simulink model "manul_model_stage15_complete_pre_engineering_20260816"  (R2025a)
settings: Solver=ode3  StartTime=0.0  StopTime=0.3  FixedStep=Ts_power  RelTol=1e-3
InitFcn:
  | run('D:/PV_MPPT/PV_ESS_MPC_Manul_Reproduction/experiments/stage15_bus_stability_20260814/pvess_stage15_busfix_init.m')
values from neighbouring files (symbols this model uses):
  Ad_mpvc = expm(A_mpvc*Ts_mpc)    [pvess_beginner_init_baseline.m]    (also in pvess_stage15_busfix_init.m; pvess_stage15_busfix_init_pre_cpl_20260817.m; pvess_stage15_busfix_init_pre_engineering_20260816.m; pvess_stage15_busfix_init_pre_gridpi_tuning_20260817.m)
  Bd_mpvc = A_mpvc\((Ad_mpvc-eye(2))*B_mpvc)    [pvess_beginner_init_baseline.m]    (also in pvess_stage15_busfix_init.m; pvess_stage15_busfix_init_pre_cpl_20260817.m; pvess_stage15_busfix_init_pre_engineering_20260816.m; pvess_stage15_busfix_init_pre_gridpi_tuning_20260817.m)
  Cdc = 18e-3    (= 0.018)    [pvess_beginner_init_baseline.m]    (also in pvess_stage15_busfix_init.m; pvess_stage15_busfix_init_pre_cpl_20260817.m; pvess_stage15_busfix_init_pre_engineering_20260816.m; pvess_stage15_busfix_init_pre_gridpi_tuning_20260817.m)
  Cpv = 10e-3    (= 0.01)    [pvess_beginner_init_baseline.m]    (also in pvess_stage15_busfix_init.m; pvess_stage15_busfix_init_pre_cpl_20260817.m; pvess_stage15_busfix_init_pre_engineering_20260816.m; pvess_stage15_busfix_init_pre_gridpi_tuning_20260817.m)
  Db0 = 1 - V_bat_nom/Vdc_ref    (= 0.75)    [pvess_beginner_init_baseline.m]    (also in pvess_stage15_busfix_init.m; pvess_stage15_busfix_init_pre_cpl_20260817.m; pvess_stage15_busfix_init_pre_engineering_20260816.m; pvess_stage15_busfix_init_pre_gridpi_tuning_20260817.m)
  Db_max = 0.95    [pvess_beginner_init_baseline.m]    (also in pvess_stage15_busfix_init.m; pvess_stage15_busfix_init_pre_cpl_20260817.m; pvess_stage15_busfix_init_pre_engineering_20260816.m; pvess_stage15_busfix_init_pre_gridpi_tuning_20260817.m)
  Db_min = 0.05    [pvess_beginner_init_baseline.m]    (also in pvess_stage15_busfix_init.m; pvess_stage15_busfix_init_pre_cpl_20260817.m; pvess_stage15_busfix_init_pre_engineering_20260816.m; pvess_stage15_busfix_init_pre_gridpi_tuning_20260817.m)
  Dpv0 = 1 - 547/Vdc_ref    (= 0.544166666667)    [pvess_beginner_init_baseline.m]    (also in pvess_stage15_busfix_init.m; pvess_stage15_busfix_init_pre_cpl_20260817.m; pvess_stage15_busfix_init_pre_engineering_20260816.m; pvess_stage15_busfix_init_pre_gridpi_tuning_20260817.m)
  Dpv_curtail_bias = 0.506    [pvess_stage15_busfix_init.m]    (also in pvess_stage15_busfix_init_pre_cpl_20260817.m; pvess_stage15_busfix_init_pre_engineering_20260816.m; pvess_stage15_busfix_init_pre_gridpi_tuning_20260817.m)
  Dpv_max = 0.75    [pvess_beginner_init_baseline.m]    (also in pvess_stage15_busfix_init.m; pvess_stage15_busfix_init_pre_cpl_20260817.m; pvess_stage15_busfix_init_pre_engineering_20260816.m; pvess_stage15_busfix_init_pre_gridpi_tuning_20260817.m)
  Dpv_min = 0.35    [pvess_beginner_init_baseline.m]    (also in pvess_stage15_busfix_init.m; pvess_stage15_busfix_init_pre_cpl_20260817.m; pvess_stage15_busfix_init_pre_engineering_20260816.m; pvess_stage15_busfix_init_pre_gridpi_tuning_20260817.m)
  Dpv_slew_down = -5.0    (= -5)    [pvess_stage15_busfix_init.m]    (also in pvess_stage15_busfix_init_pre_cpl_20260817.m; pvess_stage15_busfix_init_pre_engineering_20260816.m; pvess_stage15_busfix_init_pre_gridpi_tuning_20260817.m)
  Dpv_slew_up = 1.0    (= 1)    [pvess_stage15_busfix_init.m]    (also in pvess_stage15_busfix_init_pre_cpl_20260817.m; pvess_stage15_busfix_init_pre_engineering_20260816.m; pvess_stage15_busfix_init_pre_gridpi_tuning_20260817.m)
  Dpv_step = 2e-4    (= 0.0002)    [pvess_beginner_init_baseline.m]    (also in pvess_stage15_busfix_init.m; pvess_stage15_busfix_init_pre_cpl_20260817.m; pvess_stage15_busfix_init_pre_engineering_20260816.m; pvess_stage15_busfix_init_pre_gridpi_tuning_20260817.m)
  eps_dI = 1e-3    (= 0.001)    [pvess_beginner_init_baseline.m]    (also in pvess_stage15_busfix_init.m; pvess_stage15_busfix_init_pre_cpl_20260817.m; pvess_stage15_busfix_init_pre_engineering_20260816.m; pvess_stage15_busfix_init_pre_gridpi_tuning_20260817.m)
  eps_dV = 1e-3    (= 0.001)    [pvess_beginner_init_baseline.m]    (also in pvess_stage15_busfix_init.m; pvess_stage15_busfix_init_pre_cpl_20260817.m; pvess_stage15_busfix_init_pre_engineering_20260816.m; pvess_stage15_busfix_init_pre_gridpi_tuning_20260817.m)
  eps_inc = 1e-4    (= 0.0001)    [pvess_beginner_init_baseline.m]    (also in pvess_stage15_busfix_init.m; pvess_stage15_busfix_init_pre_cpl_20260817.m; pvess_stage15_busfix_init_pre_engineering_20260816.m; pvess_stage15_busfix_init_pre_gridpi_tuning_20260817.m)
  f_grid = 50    [pvess_beginner_init_baseline.m]    (also in pvess_stage15_busfix_init.m; pvess_stage15_busfix_init_pre_cpl_20260817.m; pvess_stage15_busfix_init_pre_engineering_20260816.m; pvess_stage15_busfix_init_pre_gridpi_tuning_20260817.m)
  freq_threshold = 0.15    [pvess_beginner_init_baseline.m]    (also in pvess_stage15_busfix_init.m; pvess_stage15_busfix_init_pre_cpl_20260817.m; pvess_stage15_busfix_init_pre_engineering_20260816.m; pvess_stage15_busfix_init_pre_gridpi_tuning_20260817.m)
  Ibat_curtail_release = -0.8*Ibat_max    (= -1333.33333333)    [pvess_stage15_busfix_init.m]    (also in pvess_stage15_busfix_init_pre_cpl_20260817.m; pvess_stage15_busfix_init_pre_engineering_20260816.m; pvess_stage15_busfix_init_pre_gridpi_tuning_20260817.m)
  Ibat_max = P_bat_rated/V_bat_nom    (= 1666.66666667)    [pvess_beginner_init_baseline.m]    (also in pvess_stage15_busfix_init.m; pvess_stage15_busfix_init_pre_cpl_20260817.m; pvess_stage15_busfix_init_pre_engineering_20260816.m; pvess_stage15_busfix_init_pre_gridpi_tuning_20260817.m)
  K_bat_sign = 1    [pvess_beginner_init_baseline.m]    (also in pvess_stage15_busfix_init.m; pvess_stage15_busfix_init_pre_cpl_20260817.m; pvess_stage15_busfix_init_pre_engineering_20260816.m; pvess_stage15_busfix_init_pre_gridpi_tuning_20260817.m)
  K_grid_sign = -1    [pvess_beginner_init_baseline.m]    (also in pvess_stage15_busfix_init.m; pvess_stage15_busfix_init_pre_cpl_20260817.m; pvess_stage15_busfix_init_pre_engineering_20260816.m; pvess_stage15_busfix_init_pre_gridpi_tuning_20260817.m)
  Ki_dc = 3.40748e5    (= 340748)    [pvess_beginner_init_baseline.m]    (also in pvess_stage15_busfix_init.m = 2131834.55064; pvess_stage15_busfix_init_pre_cpl_20260817.m; pvess_stage15_busfix_init_pre_engineering_20260816.m; pvess_stage15_busfix_init_pre_gridpi_tuning_20260817.m)
  Kii_bat = 0.150    (= 0.15)    [pvess_beginner_init_baseline.m]    (also in pvess_stage15_busfix_init.m = 0.05; pvess_stage15_busfix_init_pre_cpl_20260817.m = 0.05; pvess_stage15_busfix_init_pre_engineering_20260816.m = 0.05; pvess_stage15_busfix_init_pre_gridpi_tuning_20260817.m = 0.05)
  Kiv_bat = 650    [pvess_beginner_init_baseline.m]    (also in pvess_stage15_busfix_init.m; pvess_stage15_busfix_init_pre_cpl_20260817.m; pvess_stage15_busfix_init_pre_engineering_20260816.m; pvess_stage15_busfix_init_pre_gridpi_tuning_20260817.m)
  Kp_dc = 3836.125    [pvess_beginner_init_baseline.m]    (also in pvess_stage15_busfix_init.m = 2*zeta_dc*(2*pi*f_bw_dc)*Cdc*Vdc_ref; pvess_stage15_busfix_init_pre_cpl_20260817.m; pvess_stage15_busfix_init_pre_engineering_20260816.m; pvess_stage15_busfix_init_pre_gridpi_tuning_20260817.m)
  Kp_pv_curtail = 5e-5    (= 5e-05)    [pvess_stage15_busfix_init.m]    (also in pvess_stage15_busfix_init_pre_cpl_20260817.m; pvess_stage15_busfix_init_pre_engineering_20260816.m; pvess_stage15_busfix_init_pre_gridpi_tuning_20260817.m)
  Kpi_bat = 100e-3    (= 0.1)    [pvess_beginner_init_baseline.m]    (also in pvess_stage15_busfix_init.m = 0.005; pvess_stage15_busfix_init_pre_cpl_20260817.m = 0.005; pvess_stage15_busfix_init_pre_engineering_20260816.m = 0.005; pvess_stage15_busfix_init_pre_gridpi_tuning_20260817.m = 0.005)
  Kpv_bat = 4    [pvess_beginner_init_baseline.m]    (also in pvess_stage15_busfix_init.m; pvess_stage15_busfix_init_pre_cpl_20260817.m; pvess_stage15_busfix_init_pre_engineering_20260816.m; pvess_stage15_busfix_init_pre_gridpi_tuning_20260817.m)
  lambda_mppc = 0.001    [pvess_beginner_init_baseline.m]    (also in pvess_stage15_busfix_init.m; pvess_stage15_busfix_init_pre_cpl_20260817.m; pvess_stage15_busfix_init_pre_engineering_20260816.m; pvess_stage15_busfix_init_pre_gridpi_tuning_20260817.m)
  lambda_mpvc = 3e-6    (= 3e-06)    [pvess_beginner_init_baseline.m]    (also in pvess_stage15_busfix_init.m; pvess_stage15_busfix_init_pre_cpl_20260817.m; pvess_stage15_busfix_init_pre_engineering_20260816.m; pvess_stage15_busfix_init_pre_gridpi_tuning_20260817.m)
  Lbat = 11.25e-3    (= 0.01125)    [pvess_beginner_init_baseline.m]    (also in pvess_stage15_busfix_init.m = 0.0005; pvess_stage15_busfix_init_pre_cpl_20260817.m = 0.0005; pvess_stage15_busfix_init_pre_engineering_20260816.m = 0.0005; pvess_stage15_busfix_init_pre_gridpi_tuning_20260817.m = 0.0005)
  Lf = 0.6e-3    (= 0.0006)    [pvess_beginner_init_baseline.m]    (also in pvess_stage15_busfix_init.m; pvess_stage15_busfix_init_pre_cpl_20260817.m; pvess_stage15_busfix_init_pre_engineering_20260816.m; pvess_stage15_busfix_init_pre_gridpi_tuning_20260817.m)
  Lpv = 0.8e-3    (= 0.0008)    [pvess_beginner_init_baseline.m]    (also in pvess_stage15_busfix_init.m; pvess_stage15_busfix_init_pre_cpl_20260817.m; pvess_stage15_busfix_init_pre_engineering_20260816.m; pvess_stage15_busfix_init_pre_gridpi_tuning_20260817.m)
  m_var = 4e6    (= 4000000)    [pvess_beginner_init_baseline.m]    (also in pvess_stage15_busfix_init.m; pvess_stage15_busfix_init_pre_cpl_20260817.m; pvess_stage15_busfix_init_pre_engineering_20260816.m; pvess_stage15_busfix_init_pre_gridpi_tuning_20260817.m)
  N_ems_fast_avg = 100    [pvess_beginner_init_baseline.m]    (also in pvess_stage15_busfix_init.m; pvess_stage15_busfix_init_pre_cpl_20260817.m; pvess_stage15_busfix_init_pre_engineering_20260816.m; pvess_stage15_busfix_init_pre_gridpi_tuning_20260817.m)
  omega_grid = 2*pi*f_grid    (= 314.159265359)    [pvess_beginner_init_baseline.m]    (also in pvess_stage15_busfix_init.m; pvess_stage15_busfix_init_pre_cpl_20260817.m; pvess_stage15_busfix_init_pre_engineering_20260816.m; pvess_stage15_busfix_init_pre_gridpi_tuning_20260817.m)
  P_base_mpc = 2e6    (= 2000000)    [pvess_beginner_init_baseline.m]    (also in pvess_stage15_busfix_init.m; pvess_stage15_busfix_init_pre_cpl_20260817.m; pvess_stage15_busfix_init_pre_engineering_20260816.m; pvess_stage15_busfix_init_pre_gridpi_tuning_20260817.m)
  phase_threshold = 0.99863    [pvess_beginner_init_baseline.m]    (also in pvess_stage15_busfix_init.m; pvess_stage15_busfix_init_pre_cpl_20260817.m; pvess_stage15_busfix_init_pre_engineering_20260816.m; pvess_stage15_busfix_init_pre_gridpi_tuning_20260817.m)
  Pref_max = 2.2e6    (= 2200000)    [pvess_beginner_init_baseline.m]    (also in pvess_stage15_busfix_init.m; pvess_stage15_busfix_init_pre_cpl_20260817.m; pvess_stage15_busfix_init_pre_engineering_20260816.m; pvess_stage15_busfix_init_pre_gridpi_tuning_20260817.m)
  Pref_min = -2.2e6    (= -2200000)    [pvess_beginner_init_baseline.m]    (also in pvess_stage15_busfix_init.m; pvess_stage15_busfix_init_pre_cpl_20260817.m; pvess_stage15_busfix_init_pre_engineering_20260816.m; pvess_stage15_busfix_init_pre_gridpi_tuning_20260817.m)
  Q_base_mpc = 1e6    (= 1000000)    [pvess_beginner_init_baseline.m]    (also in pvess_stage15_busfix_init.m; pvess_stage15_busfix_init_pre_cpl_20260817.m; pvess_stage15_busfix_init_pre_engineering_20260816.m; pvess_stage15_busfix_init_pre_gridpi_tuning_20260817.m)
  Q_bat_Ah = 1300    [pvess_beginner_init_baseline.m]    (also in pvess_stage15_busfix_init.m; pvess_stage15_busfix_init_pre_cpl_20260817.m; pvess_stage15_busfix_init_pre_engineering_20260816.m; pvess_stage15_busfix_init_pre_gridpi_tuning_20260817.m)
  R_bat_internal = 0.02    [pvess_beginner_init_baseline.m]    (also in pvess_stage15_busfix_init.m; pvess_stage15_busfix_init_pre_cpl_20260817.m; pvess_stage15_busfix_init_pre_engineering_20260816.m; pvess_stage15_busfix_init_pre_gridpi_tuning_20260817.m)
  Rf = 0.019    [pvess_beginner_init_baseline.m]    (also in pvess_stage15_busfix_init.m; pvess_stage15_busfix_init_pre_cpl_20260817.m; pvess_stage15_busfix_init_pre_engineering_20260816.m; pvess_stage15_busfix_init_pre_gridpi_tuning_20260817.m)
  RLbat = 2e-3    (= 0.002)    [pvess_beginner_init_baseline.m]    (also in pvess_stage15_busfix_init.m; pvess_stage15_busfix_init_pre_cpl_20260817.m; pvess_stage15_busfix_init_pre_engineering_20260816.m; pvess_stage15_busfix_init_pre_gridpi_tuning_20260817.m)
  RLpv = 2e-3    (= 0.002)    [pvess_beginner_init_baseline.m]    (also in pvess_stage15_busfix_init.m; pvess_stage15_busfix_init_pre_cpl_20260817.m; pvess_stage15_busfix_init_pre_engineering_20260816.m; pvess_stage15_busfix_init_pre_gridpi_tuning_20260817.m)
  S_tr = 2.5e6    (= 2500000)    [pvess_beginner_init_baseline.m]    (also in pvess_stage15_busfix_init.m; pvess_stage15_busfix_init_pre_cpl_20260817.m; pvess_stage15_busfix_init_pre_engineering_20260816.m; pvess_stage15_busfix_init_pre_gridpi_tuning_20260817.m)
  SOC0 = 50    [pvess_beginner_init_baseline.m]    (also in pvess_stage15_busfix_init.m; pvess_stage15_busfix_init_pre_cpl_20260817.m; pvess_stage15_busfix_init_pre_engineering_20260816.m; pvess_stage15_busfix_init_pre_gridpi_tuning_20260817.m)
  SOC_max = 90    [pvess_beginner_init_baseline.m]    (also in pvess_stage15_busfix_init.m; pvess_stage15_busfix_init_pre_cpl_20260817.m; pvess_stage15_busfix_init_pre_engineering_20260816.m; pvess_stage15_busfix_init_pre_gridpi_tuning_20260817.m)
  SOC_min = 10    [pvess_beginner_init_baseline.m]    (also in pvess_stage15_busfix_init.m; pvess_stage15_busfix_init_pre_cpl_20260817.m; pvess_stage15_busfix_init_pre_engineering_20260816.m; pvess_stage15_busfix_init_pre_gridpi_tuning_20260817.m)
  sync_hold = 0.1    [pvess_beginner_init_baseline.m]    (also in pvess_stage15_busfix_init.m; pvess_stage15_busfix_init_pre_cpl_20260817.m; pvess_stage15_busfix_init_pre_engineering_20260816.m; pvess_stage15_busfix_init_pre_gridpi_tuning_20260817.m)
  T_ac_step = 0.2    [pvess_beginner_init_baseline.m]    (also in pvess_stage15_busfix_init.m = 0.5; pvess_stage15_busfix_init_pre_cpl_20260817.m = 0.5; pvess_stage15_busfix_init_pre_engineering_20260816.m = 0.5; pvess_stage15_busfix_init_pre_gridpi_tuning_20260817.m = 0.5)
  T_grid_connect = 1.6    [pvess_beginner_init_baseline.m]    (also in pvess_stage15_busfix_init.m; pvess_stage15_busfix_init_pre_cpl_20260817.m; pvess_stage15_busfix_init_pre_engineering_20260816.m; pvess_stage15_busfix_init_pre_gridpi_tuning_20260817.m)
  T_grid_dip = 3.5    [pvess_beginner_init_baseline.m]    (also in pvess_stage15_busfix_init.m; pvess_stage15_busfix_init_pre_cpl_20260817.m; pvess_stage15_busfix_init_pre_engineering_20260816.m; pvess_stage15_busfix_init_pre_gridpi_tuning_20260817.m)
  T_sync = 1.4    [pvess_beginner_init_baseline.m]    (also in pvess_stage15_busfix_init.m; pvess_stage15_busfix_init_pre_cpl_20260817.m; pvess_stage15_busfix_init_pre_engineering_20260816.m; pvess_stage15_busfix_init_pre_gridpi_tuning_20260817.m)
  Ts_bat_ctrl = 100e-6    (= 0.0001)    [pvess_beginner_init_baseline.m]    (also in pvess_stage15_busfix_init.m; pvess_stage15_busfix_init_pre_cpl_20260817.m; pvess_stage15_busfix_init_pre_engineering_20260816.m; pvess_stage15_busfix_init_pre_gridpi_tuning_20260817.m)
  Ts_ems = 1e-3    (= 0.001)    [pvess_beginner_init_baseline.m]    (also in pvess_stage15_busfix_init.m; pvess_stage15_busfix_init_pre_cpl_20260817.m; pvess_stage15_busfix_init_pre_engineering_20260816.m; pvess_stage15_busfix_init_pre_gridpi_tuning_20260817.m)
  Ts_mpc = 1/20e3    (= 5e-05)    [pvess_beginner_init_baseline.m]    (also in pvess_stage15_busfix_init.m; pvess_stage15_busfix_init_pre_cpl_20260817.m; pvess_stage15_busfix_init_pre_engineering_20260816.m; pvess_stage15_busfix_init_pre_gridpi_tuning_20260817.m)
  Ts_mppt = 1e-3    (= 0.001)    [pvess_beginner_init_baseline.m]    (also in pvess_stage15_busfix_init.m; pvess_stage15_busfix_init_pre_cpl_20260817.m; pvess_stage15_busfix_init_pre_engineering_20260816.m; pvess_stage15_busfix_init_pre_gridpi_tuning_20260817.m)
  Ts_power = 2e-6    (= 2e-06)    [pvess_beginner_init_baseline.m]    (also in pvess_stage15_busfix_init.m; pvess_stage15_busfix_init_pre_cpl_20260817.m; pvess_stage15_busfix_init_pre_engineering_20260816.m; pvess_stage15_busfix_init_pre_gridpi_tuning_20260817.m)
  Ts_soc = 1e-4    (= 0.0001)    [pvess_beginner_init_baseline.m]    (also in pvess_stage15_busfix_init.m; pvess_stage15_busfix_init_pre_cpl_20260817.m; pvess_stage15_busfix_init_pre_engineering_20260816.m; pvess_stage15_busfix_init_pre_gridpi_tuning_20260817.m)
  V_bat_nom = 300    [pvess_beginner_init_baseline.m]    (also in pvess_stage15_busfix_init.m; pvess_stage15_busfix_init_pre_cpl_20260817.m; pvess_stage15_busfix_init_pre_engineering_20260816.m; pvess_stage15_busfix_init_pre_gridpi_tuning_20260817.m)
  V_tr_hv = 25e3    (= 25000)    [pvess_beginner_init_baseline.m]    (also in pvess_stage15_busfix_init.m; pvess_stage15_busfix_init_pre_cpl_20260817.m; pvess_stage15_busfix_init_pre_engineering_20260816.m; pvess_stage15_busfix_init_pre_gridpi_tuning_20260817.m)
  V_tr_lv = Vac_ll    (= 690)    [pvess_beginner_init_baseline.m]    (also in pvess_stage15_busfix_init.m; pvess_stage15_busfix_init_pre_cpl_20260817.m; pvess_stage15_busfix_init_pre_engineering_20260816.m; pvess_stage15_busfix_init_pre_gridpi_tuning_20260817.m)
  Vac_phase_peak = sqrt(2)*Vac_ll/sqrt(3)    [pvess_beginner_init_baseline.m]    (also in pvess_stage15_busfix_init.m; pvess_stage15_busfix_init_pre_cpl_20260817.m; pvess_stage15_busfix_init_pre_engineering_20260816.m; pvess_stage15_busfix_init_pre_gridpi_tuning_20260817.m)
  Vdc_curtail_off = 1185    [pvess_stage15_busfix_init.m]    (also in pvess_stage15_busfix_init_pre_cpl_20260817.m; pvess_stage15_busfix_init_pre_engineering_20260816.m; pvess_stage15_busfix_init_pre_gridpi_tuning_20260817.m)
  Vdc_curtail_on = 1220    [pvess_stage15_busfix_init.m]    (also in pvess_stage15_busfix_init_pre_cpl_20260817.m; pvess_stage15_busfix_init_pre_engineering_20260816.m; pvess_stage15_busfix_init_pre_gridpi_tuning_20260817.m)
  Vdc_ref = 1200    [pvess_beginner_init_baseline.m]    (also in pvess_stage15_busfix_init.m; pvess_stage15_busfix_init_pre_cpl_20260817.m; pvess_stage15_busfix_init_pre_engineering_20260816.m; pvess_stage15_busfix_init_pre_gridpi_tuning_20260817.m)
  Vf_diode = 1.0    (= 1)    [pvess_beginner_init_baseline.m]    (also in pvess_stage15_busfix_init.m; pvess_stage15_busfix_init_pre_cpl_20260817.m; pvess_stage15_busfix_init_pre_engineering_20260816.m; pvess_stage15_busfix_init_pre_gridpi_tuning_20260817.m)
  Vpv0 = 547    [pvess_beginner_init_baseline.m]    (also in pvess_stage15_busfix_init.m; pvess_stage15_busfix_init_pre_cpl_20260817.m; pvess_stage15_busfix_init_pre_engineering_20260816.m; pvess_stage15_busfix_init_pre_gridpi_tuning_20260817.m)
  Vsync_threshold = 10    [pvess_beginner_init_baseline.m]    (also in pvess_stage15_busfix_init.m; pvess_stage15_busfix_init_pre_cpl_20260817.m; pvess_stage15_busfix_init_pre_engineering_20260816.m; pvess_stage15_busfix_init_pre_gridpi_tuning_20260817.m)
undefined symbols (not defined in the file or in its folder): DiscIntNeverNeededParam, dspblkCoreblockFVToolHelper, gcbh, Ion, Kt_dc, Lithium
libraries: dspstat3 x10, simulink x9, spsBreakerLib x5, spsCurrentMeasurementLib x4, slpidlib x3, spsThreePhaseVIMeasurementLib x3, eeRmsMeasurement x3, spsThreePhaseParallelRLCLoadLib x3, spsThreePhaseBreakerLib x3, spsParallelRLCBranchLib x2, spsVariableResistorLib x2, spsThreePhaseSeriesRLCBranchLib x2
(part 1 of 2)
settings Model: Creator=Limingyu  LastModifiedBy=Administrator

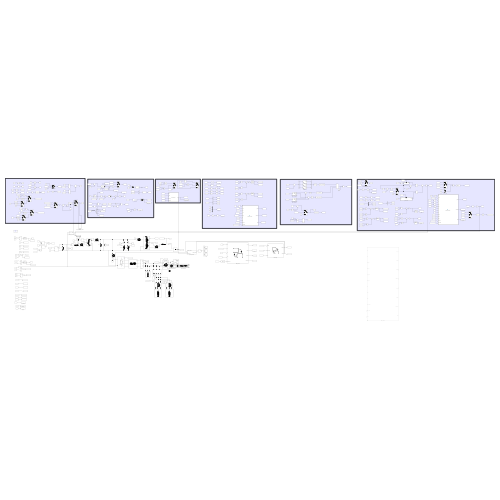
[thumbnail: Simulink's stored preview of the top-level diagram]
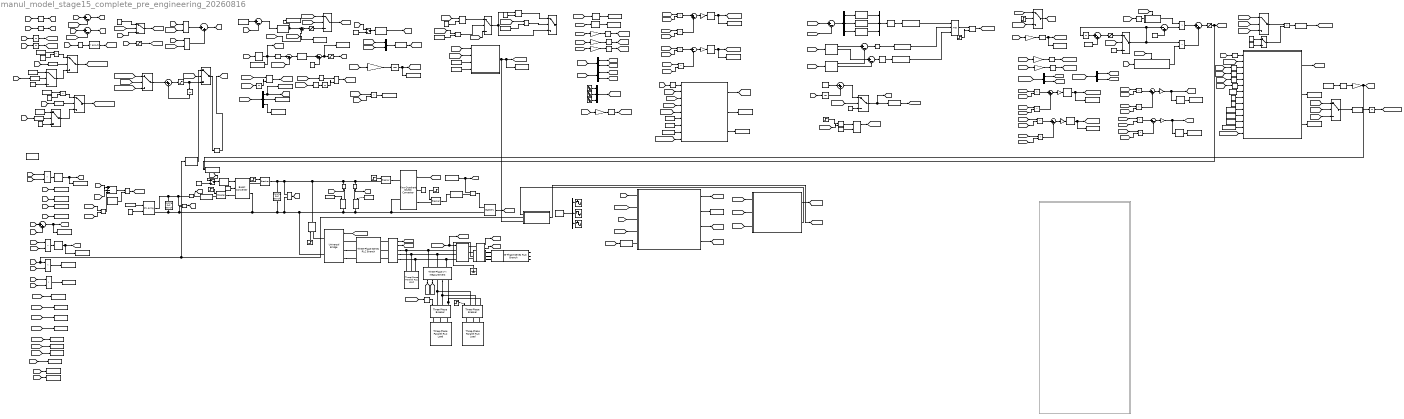
== system manul_model_stage15_complete_pre_engineering_20260816 ==
  note: 并网许可与保存控制
  note: MPPC
  note: MPVC
  note: SOC保护
  note: 电池双环控制
  note: MPPT algorithm
  AC_load_Step : Step  Time=T_ac_step  SampleTime=0
  AND{,1..2,4} (4 alike) : Logic  IconShape=distinctive  AllPortsSameDT=off  OutDataTypeStr=boolean
  AND3 : Logic  Inputs=3  IconShape=distinctive  AllPortsSameDT=off  OutDataTypeStr=boolean
  A_phase : Sin  Amplitude=0.9  Frequency=2*pi*f_grid  SampleTime=Ts_power
  Abs : Abs  SaturateOnIntegerOverflow=off
  Abs2 : Abs  SaturateOnIntegerOverflow=off
  B_phase : Sin  Amplitude=0.9  Frequency=2*pi*f_grid  Phase=-2*pi/3  SampleTime=Ts_power
  Battery : spsBatteryLib/Battery  BatType=Lithium-Ion  NomV=V_bat_nom  NomQ=Q_bat_Ah  SOC=SOC0  Batt_Tr=30  PresetModel=off  MaxQ=1300  MinV=270  FullV=330  Dis_rate=565.2174  R=R_bat_internal  Normal_OP=1175.6522  expZone="[324.1158      63.86957]"
  Battery DC Isolator : spsBreakerLib/Breaker  InitialState=0  SwitchingTimes="[1/60  5/60]"  External=on  BreakerResistance=0.001  SnubberResistance=1e6  SnubberCapacitance=inf  Measurements=None  MoreParameters=on  NoBreakLoop=off
  Battery Isolato : spsBreakerLib/Breaker  InitialState=0  SwitchingTimes="[1/60  5/60]"  External=on  BreakerResistance=0.001  SnubberResistance=1e6  SnubberCapacitance=inf  Measurements=None  MoreParameters=on  NoBreakLoop=off
  Bias : Bias  Bias=-1  SaturateOnIntegerOverflow=off
  Breaker : spsBreakerLib/Breaker  InitialState=0  SwitchingTimes="[1/60  5/60]"  External=on  BreakerResistance=0.01  SnubberResistance=1e6  SnubberCapacitance=inf  Measurements=None  MoreParameters=on  NoBreakLoop=off
  Bus Selector : BusSelector  OutputSignals=Voltage (V),Current (A),SOC (%)
  C_phase : Sin  Amplitude=0.9  Frequency=2*pi*f_grid  Phase=2*pi/3  SampleTime=Ts_power
  C_pv : spsParallelRLCBranchLib/Parallel RLC Branch  LConnTagsString=a  RConnTagsString=__new0  BranchType=C  Resistance=1  Inductance=1e-3  SetiL0=off  InitialCurrent=0  Capacitance=Cpv  Setx0=on  InitialVoltage=Vpv0  Measurements=None
  Cdc : spsParallelRLCBranchLib/Parallel RLC Branch  LConnTagsString=a  RConnTagsString=__new0  BranchType=C  Resistance=1  Inductance=1e-3  SetiL0=off  InitialCurrent=0  Capacitance=Cdc  Setx0=on  InitialVoltage=Vdc0  Measurements=None
  Compare To Constant : simulink/Logic and Bit Operations/Compare To Constant  relop=>  const=eps_inc  OutDataTypeStr=boolean
  Compare To Constant1 : simulink/Logic and Bit Operations/Compare To Constant  relop=<  const=eps_dV  OutDataTypeStr=boolean
  Compare To Constant2 : simulink/Logic and Bit Operations/Compare To Constant  relop=<  const=-eps_inc  OutDataTypeStr=boolean
  Compare To Constant3 : simulink/Logic and Bit Operations/Compare To Constant  relop=>  const=eps_dI  OutDataTypeStr=boolean
  Compare To Constant4 : simulink/Logic and Bit Operations/Compare To Constant  relop=<  const=-eps_dI  OutDataTypeStr=boolean
  Compare To Constant5 : simulink/Logic and Bit Operations/Compare To Constant  relop=<=  const=Vsync_threshold  OutDataTypeStr=boolean
  Compare To Constant6 : simulink/Logic and Bit Operations/Compare To Constant  relop=<=  const=freq_threshold  OutDataTypeStr=boolean
  Compare To Constant7 : simulink/Logic and Bit Operations/Compare To Constant  relop=>=  const=phase_threshold  OutDataTypeStr=boolean
  Compare To Constant8 : simulink/Logic and Bit Operations/Compare To Constant  relop=>=  const=sync_hold  OutDataTypeStr=boolean
  Constant : Constant  Value=V_bat_nom
  Constant1 : Constant  Value=25
  Constant10 : Constant  Value=-1
  Constant{5,7..8,11} (4 alike) : Constant  Value=Dpv_step
  Constant{3,9,12,14,22,26..27,32,42} (9 alike) : Constant  Value=0
  Constant13 : Constant  Value=Db0
  Constant16 : Constant  Value=Db0
  Constant17 : Constant  Value=Ts_mpc
  Constant2 : Constant  Value=Dpv0
  Constant20 : Constant  Value=SOC_max
  Constant21 : Constant  Value=SOC_min
  Constant23 : Constant  Value=SOC_min
  Constant24 : Constant  Value=SOC_max
  Constant25 : Constant  Value=lambda_mpvc
  Constant28 : Constant  Value=Ad_mpvc
  Constant29 : Constant  Value=Bd_mpvc
  Constant30 : Constant
  Constant33 : Constant  Value=Ts_mpc
  Constant34 : Constant  Value=Lf
  Constant35 : Constant  Value=omega_grid
  Constant36 : Constant  Value=Rf
  Constant37 : Constant  Value=lambda_mppc
  Constant38 : Constant  Value=P_base_mpc
  Constant39 : Constant  Value=Q_base_mpc
  Constant4 : Constant
  Constant40 : Constant  Value=0  OutDataTypeStr=boolean
  Constant41 : Constant  Value=3.333e-4
  Constant43 : Constant
  Constant6 : Constant  Value=-1
  Current Measurement{,1..3} (4 alike) : spsCurrentMeasurementLib/Current Measurement  PhasorSimulation=off  OutputType=Complex  PSBequivalent=0
  DC_load1 : spsVariableResistorLib/Variable Resistor  Rabsmin=0.2
      settings: LibrarySourceBlock=sps_lib/Passives/Variable Resistor
  DC_load2 : spsVariableResistorLib/Variable Resistor  Rabsmin=0.2
      settings: LibrarySourceBlock=sps_lib/Passives/Variable Resistor
  DC_output_isolator : spsBreakerLib/Breaker  InitialState=0  SwitchingTimes="[1/60  5/60]"  External=on  BreakerResistance=0.001  SnubberResistance=1e6  SnubberCapacitance=inf  Measurements=None  MoreParameters=on  NoBreakLoop=off
  D_bat : ToWorkspace  VariableName=D_bat  SaveFormat=Timeseries  SampleTime=-1
  Data Type Conversion : DataTypeConversion  OutDataTypeStr=double  SaturateOnIntegerOverflow=off  RndMeth=Floor
  Data Type Conversion1 : DataTypeConversion  OutDataTypeStr=double  SaturateOnIntegerOverflow=off  RndMeth=Floor
  Data Type Conversion2 : DataTypeConversion  OutDataTypeStr=double  SaturateOnIntegerOverflow=off  RndMeth=Floor
  Demux{,1..3} (4 alike) : Demux  Outputs=2
  Demux4 : Demux  Outputs=3
  Discrete PID Controller : slpidlib/PID Controller  Controller=PI  Form=Parallel  TimeDomain=Discrete-time  UseExternalTs=off  SampleTime=Ts_bat_ctrl  IntegratorMethod=Forward Euler  FilterMethod=Forward Euler  ControllerParametersSource=internal  P=Kpi_bat  I=Kii_bat  UseKiTs=off  D=0  UseExternalDerivativeSource=off  N=100  UseFilter=on  TunerSelectOption=Transfer Function Based (PID Tuner App)  InitialConditionSource=internal  InitialConditionForIntegrator=0  InitialConditionForFilter=0  DifferentiatorICPrevScaledInput=0  ExternalReset=none  TrackingMode=off  Kt=1  LimitOutput=on  SatLimitsSource=internal  UpperSaturationLimit=0.25  LowerSaturationLimit=-0.25  LinearizeAsGain=off  AntiWindupMode=clamping  Kb=1  LimitIntegrator=off  UpperIntegratorSaturationLimit=inf  LowerIntegratorSaturationLimit=-inf  POutMin=[]  POutMax=[]  IOutMin=[]  IOutMax=[]  DOutMin=[]  DOutMax=[]  NOutMin=[]  NOutMax=[]  SumOutMin=[]  SumOutMax=[]  SaturationOutMin=[]  SaturationOutMax=[]  PParamMin=[]  PParamMax=[]  IParamMin=[]  IParamMax=[]  DParamMin=[]  DParamMax=[]  NParamMin=[]  NParamMax=[]  KbParamMin=[]  KbParamMax=[]  KtParamMin=[]  KtParamMax=[]  KbOutMin=[]  KbOutMax=[]  KtOutMin=[]  KtOutMax=[]  IntegratorOutMin=[]  IntegratorOutMax=[]  FilterOutMin=[]  FilterOutMax=[]  SumI1OutMin=[]  SumI1OutMax=[]  SumI2OutMin=[]  SumI2OutMax=[]  SumI3OutMin=[]  SumI3OutMax=[]  SumI4OutMin=[]  SumI4OutMax=[]  SumDOutMin=[]  SumDOutMax=[]  DifferentiatorOutMin=[]  DifferentiatorOutMax=[]  FilterDiffOutCoefMin=[]  FilterDiffOutCoefMax=[]  ReciprocalOutMin=[]  ReciprocalOutMax=[]  SumDenOutMin=[]  SumDenOutMax=[]  SumNumOutMin=[]  SumNumOutMax=[]  DivideOutMin=[]  DivideOutMax=[]  UdiffTsProdOutMin=[]  UdiffTsProdOutMax=[]  NTsProdOutMin=[]  NTsProdOutMax=[]  UintegralTsProdOutMin=[]  UintegralTsProdOutMax=[]  UngainTsProdOutMin=[]  UngainTsProdOutMax=[]  ClampingZeroOutDataTypeStr=Inherit: Inherit via back propagation  ClampingZeroOutMin=[]  ClampingZeroOutMax=[]  FilterDenConstantOutDataTypeStr=Inherit: Inherit via back propagation  FilterDenConstantOutMin=[]  FilterDenConstantOutMax=[]  PCopyOutDataTypeStr=Inherit: Inherit via back propagation  PCopyOutMin=[]  PCopyOutMax=[]  NCopyOutDataTypeStr=Inherit: Inherit via back propagation  NCopyOutMin=[]  NCopyOutMax=[]  IntegratorContinuousStateAttributes=''  IntegratorStateMustResolveToSignalObject=off  IntegratorRTWStateStorageClass=Auto  FilterContinuousStateAttributes=''  FilterStateMustResolveToSignalObject=off  FilterRTWStateStorageClass=Auto  ParallelPVariant=InternalParameters  IdealPVariant=Disabled  IVariant=InternalParameters  DVariant=Disabled  IntegratorVariant=Discrete  SatVariant=Enabled  AWVariant=DiscClampingParallel  PCopyVariant=Disabled  TRVariant=Disabled  FdbkBlocksVariant=Forward  IdealPFdbkVariant=Disabled  SatFdbkVariant=Disabled  DerivativeFilterVariant=Disabled  NVariant=Disabled  NCopyVariant=Disabled_SignalSpec  FilterICVariant=Disabled  IntegratorICVariant=InternalICs  ExternalResetVariant=Disabled  TRSumVariant=Passthrough  SumFdbkVariant=Disabled  SumVariant=Sum_PI  TsampFilterVariant=InternalTs  TsampNgainVariant=Passthrough  TsampIntegralVariant=Disabled_SignalSpec  ExternalSaturationOutDataTypeStr=Inherit: Same as second input  DerivativeSourceVariant=Disabled  PreIntVariant=InternalPreInt
      settings: LibrarySourceBlock=simulink/Discrete/Discrete PID Controller
  Discrete-Time Integrator : DiscreteIntegrator  InitialCondition=SOC0  SampleTime=Ts_bat_ctrl  LimitOutput=on  UpperSaturationLimit=100  LowerSaturationLimit=0  ICPrevOutput=DiscIntNeverNeededParam  ICPrevScaledInput=DiscIntNeverNeededParam
  Divide : Product  Inputs=*/
  Divide1 : Product  Inputs=*/
  Divide2 : Product  Inputs=*/
  Dot Product : DotProduct  OutDataTypeStr=Inherit: Inherit via internal rule
  Dpv : ToWorkspace  VariableName=Dpv  SaveFormat=Timeseries  SampleTime=-1
  EMS_Controller : Subsystem  Commented=on
  EMS_flowchart : Stateflow chart  TreatAsAtomicUnit=on
  From Workspace : FromWorkspace  VariableName=Rdc1_profile  OutputAfterFinalValue=Holding final value
  From Workspace1 : FromWorkspace  VariableName=Rdc2_profile  OutputAfterFinalValue=Holding final value
  From Workspace2 : FromWorkspace  VariableName=G_profile  OutputAfterFinalValue=Holding final value
  Gain : Gain  Gain=m_var
  Gain{1..3,6..7,9..10} (7 alike) : Gain  Gain=[2/3 -1/3 -1/3;0 1/sqrt(3) -1/sqrt(3)]  Multiplication=Matrix(K*u)
  Gain{4..5,8,11..13} (6 alike) : Gain  Gain=3/2
  GridConnectEnable : Step  Time=T_grid_connect  SampleTime=Ts_mpc
  Grid_Equivalent_RL : spsThreePhaseSeriesRLCBranchLib/Three-Phase Series RLC Branch  LConnTagsString=A|B|C  RConnTagsString=A|B|C  BranchType=RL  Resistance=0.8929  Inductance=16.58e-3  Capacitance=1e-6  Measurements=None
  Grid_Programmable_Voltage_Source : spsThreePhaseProgrammableVoltageSourceLib/Three-Phase Programmable Voltage Source  PositiveSequence=[V_tr_hv 0 f_grid]  VariationEntity=Amplitude  VariationType=Table of time-amplitude pairs  VariationTypeAlt=Step  VariationStep=0.5  VariationRate=10  VariationMagnitude=0.3  VariationFrequency=2  VariationTiming=[1 2]  VariationPhaseA=off  Amplitudes=[1 1 0.9 0.9]  TimeValues=[0 T_grid_dip T_grid_dip+Ts_power 4]  HarmonicGeneration=off  HarmonicA=[3 0.2 -25 0]  HarmonicB=[2 0.15 35 2]  Timing="[0.05  3]"  BusType=swing  Pref=10e3  Qref=0  Qmin=-inf  Qmax=inf
  Grid_Source_Ground : spsGroundLib/Ground  LConnTagsString=a
  I_bat : ToWorkspace  VariableName=I_bat  SaveFormat=Timeseries  SampleTime=-1
  I_bat to SOC : Gain  Gain=-100/(3600*Q_bat_Ah)
  I_bat_mean : ToWorkspace  VariableName=I_bat_mean  SaveFormat=Timeseries  SampleTime=-1
  I_load_clarke : ToWorkspace  VariableName=I_load_clarke  SaveFormat=Timeseries  SampleTime=-1
  I_pv : ToWorkspace  VariableName=I_pv  SaveFormat=Timeseries  SampleTime=-1
  I_ref_ems : ToWorkspace  VariableName=I_ref_ems  SaveFormat=Timeseries  SampleTime=-1
  I_ref_protected : ToWorkspace  VariableName=I_ref_protected  SaveFormat=Timeseries  SampleTime=-1
  I_ref_raw : ToWorkspace  VariableName=I_ref_raw  SaveFormat=Timeseries  SampleTime=-1
  I_sourcebat : ToWorkspace  VariableName=I_sourcebat  SaveFormat=Timeseries  SampleTime=-1
  Iabc_L : ToWorkspace  VariableName=Iabc_L  SaveFormat=Timeseries  SampleTime=-1
  Iabc_L_rms : ToWorkspace  VariableName=Iabc_L_rms  SaveFormat=Timeseries  SampleTime=-1
  Iabc_grid : ToWorkspace  VariableName=Iabc_grid  SaveFormat=Timeseries  SampleTime=-1
  Iabc_load : ToWorkspace  VariableName=Iabc_load  SaveFormat=Timeseries  SampleTime=-1
  Idc_load : ToWorkspace  VariableName=Idc_load  SaveFormat=Timeseries  SampleTime=-1
  If_clarke : ToWorkspace  VariableName=If_clarke  SaveFormat=Timeseries  SampleTime=-1
  Jmin_MPPC : ToWorkspace  VariableName=Jmin_MPPC  SaveFormat=Timeseries  SampleTime=-1
  Jmin_mpvc : ToWorkspace  VariableName=Jmin_mpvc  SaveFormat=Timeseries  SampleTime=-1
  LC_VI : spsThreePhaseVIMeasurementLib/Three-Phase V-I Measurement  VoltageMeasurement=phase-to-ground  SetLabelV=off  LabelV=Vabc  Vpu=off  VpuLL=off  CurrentMeasurement=yes  SetLabelI=off  LabelI=Iabc  Ipu=off  Pbase=100e6  Vbase=500e3  OutputType=Complex  PhasorSimulation=off  PSBequivalent=0
  L_pv : spsSeriesRLCBranchLib/Series RLC Branch  LConnTagsString=__new0  RConnTagsString=__new0  BranchType=RL  Resistance=RLpv  Inductance=Lpv  SetiL0=off  InitialCurrent=0  Capacitance=Lpv  Setx0=on  InitialVoltage=ILpv0  Measurements=None
  Log_Pref_Command : ToWorkspace  VariableName=P_ref_cmd  SaveFormat=Timeseries
      settings: Decimation=20
  Log_Qref_Command : ToWorkspace  VariableName=Q_ref_cmd  SaveFormat=Timeseries
      settings: Decimation=20
  MATLAB Function : MATLAB Function  TreatAsAtomicUnit=on
  MATLAB Function1 : MATLAB Function  TreatAsAtomicUnit=on
  MATLAB Function2 : MATLAB Function  TreatAsAtomicUnit=on
  Manual Switch : ManualSwitch
  Manual Switch1 : ManualSwitch
  Max : MinMax  Function=max  Inputs=2
  Max1 : MinMax  Inputs=2
  MinMax1 : MinMax  Function=max
  Moving Average{,1..2,4..6,9..10} (8 alike) : dspstat3/Moving Average  Method=Sliding window  ForgettingFactorPort=off  SpecifyWindowLength=on  WindowLength=100  OverlapLength=99  AllowArbitraryInputLength=off  ForgettingFactor=0.9  SimulateUsing=Interpreted execution
  Moving Average3 : dspstat3/Moving Average  Method=Sliding window  ForgettingFactorPort=off  SpecifyWindowLength=on  WindowLength=20  OverlapLength=19  AllowArbitraryInputLength=off  ForgettingFactor=0.9  SimulateUsing=Interpreted execution
  Mux : Mux  Inputs=2
  Mux1 : Mux  Inputs=3
  Mux2 : Mux  Inputs=3
  Mux3 : Mux  Inputs=3
  NOT : Logic  Operator=NOT  IconShape=distinctive  AllPortsSameDT=off  OutDataTypeStr=boolean
  NOT1 : Logic  Operator=NOT  IconShape=distinctive  AllPortsSameDT=off  OutDataTypeStr=boolean
  NOT2 : Logic  Operator=NOT  IconShape=distinctive  AllPortsSameDT=off  OutDataTypeStr=boolean
  PI_voltage : slpidlib/PID Controller  Controller=PI  Form=Parallel  TimeDomain=Discrete-time  UseExternalTs=off  SampleTime=Ts_bat_ctrl  IntegratorMethod=Forward Euler  FilterMethod=Forward Euler  ControllerParametersSource=internal  P=Kpv_bat  I=Kiv_bat  UseKiTs=off  D=0  UseExternalDerivativeSource=off  N=100  UseFilter=on  TunerSelectOption=Transfer Function Based (PID Tuner App)  InitialConditionSource=internal  InitialConditionForIntegrator=0  InitialConditionForFilter=0  DifferentiatorICPrevScaledInput=0  ExternalReset=none  TrackingMode=off  Kt=1  LimitOutput=on  SatLimitsSource=internal  UpperSaturationLimit=Ibat_max  LowerSaturationLimit=-Ibat_max  LinearizeAsGain=off  AntiWindupMode=back-calculation  Kb=143  LimitIntegrator=off  UpperIntegratorSaturationLimit=inf  LowerIntegratorSaturationLimit=-inf  POutMin=[]  POutMax=[]  IOutMin=[]  IOutMax=[]  DOutMin=[]  DOutMax=[]  NOutMin=[]  NOutMax=[]  SumOutMin=[]  SumOutMax=[]  SaturationOutMin=[]  SaturationOutMax=[]  PParamMin=[]  PParamMax=[]  IParamMin=[]  IParamMax=[]  DParamMin=[]  DParamMax=[]  NParamMin=[]  NParamMax=[]  KbParamMin=[]  KbParamMax=[]  KtParamMin=[]  KtParamMax=[]  KbOutMin=[]  KbOutMax=[]  KtOutMin=[]  KtOutMax=[]  IntegratorOutMin=[]  IntegratorOutMax=[]  FilterOutMin=[]  FilterOutMax=[]  SumI1OutMin=[]  SumI1OutMax=[]  SumI2OutMin=[]  SumI2OutMax=[]  SumI3OutMin=[]  SumI3OutMax=[]  SumI4OutMin=[]  SumI4OutMax=[]  SumDOutMin=[]  SumDOutMax=[]  DifferentiatorOutMin=[]  DifferentiatorOutMax=[]  FilterDiffOutCoefMin=[]  FilterDiffOutCoefMax=[]  ReciprocalOutMin=[]  ReciprocalOutMax=[]  SumDenOutMin=[]  SumDenOutMax=[]  SumNumOutMin=[]  SumNumOutMax=[]  DivideOutMin=[]  DivideOutMax=[]  UdiffTsProdOutMin=[]  UdiffTsProdOutMax=[]  NTsProdOutMin=[]  NTsProdOutMax=[]  UintegralTsProdOutMin=[]  UintegralTsProdOutMax=[]  UngainTsProdOutMin=[]  UngainTsProdOutMax=[]  ClampingZeroOutDataTypeStr=Inherit: Inherit via back propagation  ClampingZeroOutMin=[]  ClampingZeroOutMax=[]  FilterDenConstantOutDataTypeStr=Inherit: Inherit via back propagation  FilterDenConstantOutMin=[]  FilterDenConstantOutMax=[]  PCopyOutDataTypeStr=Inherit: Inherit via back propagation  PCopyOutMin=[]  PCopyOutMax=[]  NCopyOutDataTypeStr=Inherit: Inherit via back propagation  NCopyOutMin=[]  NCopyOutMax=[]  IntegratorContinuousStateAttributes=''  IntegratorStateMustResolveToSignalObject=off  IntegratorRTWStateStorageClass=Auto  FilterContinuousStateAttributes=''  FilterStateMustResolveToSignalObject=off  FilterRTWStateStorageClass=Auto  ParallelPVariant=InternalParameters  IdealPVariant=Disabled  IVariant=InternalParameters  DVariant=Disabled  IntegratorVariant=Discrete  SatVariant=Enabled  AWVariant=BackCalculation  PCopyVariant=Disabled  TRVariant=Disabled  FdbkBlocksVariant=Forward  IdealPFdbkVariant=Disabled  SatFdbkVariant=Disabled  DerivativeFilterVariant=Disabled  NVariant=Disabled  NCopyVariant=Disabled_SignalSpec  FilterICVariant=Disabled  IntegratorICVariant=InternalICs  ExternalResetVariant=Disabled  TRSumVariant=Passthrough  SumFdbkVariant=Disabled  SumVariant=Sum_PI  TsampFilterVariant=InternalTs  TsampNgainVariant=Passthrough  TsampIntegralVariant=Disabled_SignalSpec  ExternalSaturationOutDataTypeStr=Inherit: Same as second input  DerivativeSourceVariant=Disabled  PreIntVariant=InternalPreInt
      settings: LibrarySourceBlock=simulink/Discrete/Discrete PID Controller
  PV Array : spsPVArrayLib/PV Array  Npar=Np_pv  Nser=Ns_pv  PlotType=array @ 25 deg.C & specified irradiances  S_vec="[ 1000  500  100 ]"  Temp_C_vec="[ 45 25  ]"  ModuleName=SunPower SPR-305E-WHT-D  PlotWhenSelected=off  Pm=305.226  Ncell=96  Voc=64.2  Isc=5.96  Vm=54.7  Im=5.58  beta_Voc_pc=-0.2727  alpha_Isc_pc=0.061745  beta_Voc=-0.17507  alpha_Isc=0.00368  IL=5.9657  I0=6.3076e-12  nI=0.94489  Rsh=393.2054  Rs=0.37428  RobustModel=off  RobustCellTemperature=313.3991  BAL=on  Tc=1e-6  Tfilter=5e-5
  PV_Curtail_Duty_Controller : Subsystem
  PV_Curtail_Protection : Subsystem
  PV_Duty_Bumpless_Transfer : RateLimiter  RisingSlewLimit=Dpv_slew_up  FallingSlewLimit=Dpv_slew_down  InitialCondition=Dpv_curtail_bias
  PWM Generator (2-Level) : spsPWMGenerator2LevelLib/PWM Generator (2-Level)  ModulatorType=Three-phase bridge (6 pulses)  ModulatorMode=Unsynchronized  Fc=3.3e3  Pc=90  nF=27  MinMax="[ -1  1 ]"  SamplingTechnique=Natural  ModulatingSignals=off  m=0.8  Freq=60  Phase=0  Ts=Ts_power  ShowCarrierOutport=off
  PWM Generator (DC-DC) : spsPWMGeneratorDCDCLib/PWM Generator (DC-DC)  Fsw=Fsw_pv  Ts=Ts_power
  PWM Generator (DC-DC)1 : spsPWMGeneratorDCDCLib/PWM Generator (DC-DC)  Fsw=Fsw_bat  Ts=Ts_power
  P_DC : ToWorkspace  VariableName=P_DC  SaveFormat=Timeseries  SampleTime=-1
  P_DC_load1 : ToWorkspace  VariableName=P_DC_load1  SaveFormat=Timeseries  SampleTime=-1
  P_DC_load2 : ToWorkspace  VariableName=P_DC_load2  SaveFormat=Timeseries  SampleTime=-1
  "P_MPPC " : ToWorkspace  VariableName=P_MPPC  SaveFormat=Timeseries  SampleTime=-1
  P_bat : ToWorkspace  VariableName=P_bat  SaveFormat=Timeseries  SampleTime=-1
  P_pv : ToWorkspace  VariableName=P_pv  SaveFormat=Timeseries  SampleTime=-1
  P_ref  occured : Subsystem  TreatAsAtomicUnit=on
  Pf_threephase : ToWorkspace  VariableName=Pf_threephase  SaveFormat=Timeseries  SampleTime=-1
  Product{,1..21} (22 alike) : Product
  ProtectionLogic : Stateflow chart  TreatAsAtomicUnit=on
  Pv_boost : spsBoostConverterLib/Boost Converter  ModelType=Switching devices  Ron=Ron_switch  Rs=1e6  Cs=inf  Vforward=[0,0]  Ron_Diode=1e-3  Rs_Diode=1e6  Cs_Diode=inf  Vf_Diode=1e-3  Rs_CurrentSource=inf  Ron_ACsource=1e-3
      settings: LibrarySourceBlock=sps_lib/Power Electronics/Boost Converter
  Pv_input_isolator : spsBreakerLib/Breaker  InitialState=0  SwitchingTimes="[1/60  5/60]"  External=on  BreakerResistance=0.001  SnubberResistance=1e6  SnubberCapacitance=inf  Measurements=None  MoreParameters=on  NoBreakLoop=off
  Q_MPPC : ToWorkspace  VariableName=Q_MPPC  SaveFormat=Timeseries  SampleTime=-1
  Qf_threephase : ToWorkspace  VariableName=Qf_threephase  SaveFormat=Timeseries  SampleTime=-1
  RMS : spsRMSLib/RMS  TrueRMS=on  Freq=50  RMSInit=398.37  Ts=Ts_power
  RMS Measurement : eeRmsMeasurement/RMS Measurement  LabelModeActiveChoice=Total  F=50  SpecifyHarmonics=off  K=[0 1 2]  Ts=Ts_mpc
      settings: LibrarySourceBlock=|
      | ee_sl_lib/Measurements/RMS
      | Measurement
  RMS Measurement1 : eeRmsMeasurement/RMS Measurement  LabelModeActiveChoice=Total  F=50  SpecifyHarmonics=off  K=[0 1 2]  Ts=Ts_mpc
      settings: LibrarySourceBlock=|
      | ee_sl_lib/Measurements/RMS
      | Measurement
  RMS Measurement2 : eeRmsMeasurement/RMS Measurement  LabelModeActiveChoice=Total  F=50  SpecifyHarmonics=off  K=[0 1 2]  Ts=Ts_mpc
      settings: LibrarySourceBlock=|
      | ee_sl_lib/Measurements/RMS
      | Measurement
  RMS1 : spsRMSLib/RMS  TrueRMS=on  Freq=50  RMSInit=398.37  Ts=Ts_power
  Relational Operator1 : RelationalOperator  OutDataTypeStr=boolean  RndMeth=Simplest  InputSameDT=off
  Relational Operator3 : RelationalOperator  Operator=<=  OutDataTypeStr=boolean  RndMeth=Simplest  InputSameDT=off
  S-R Flip-Flop : simulink_extras/Flip Flops/S-R Flip-Flop  initial_condition=0
  SOC_internal : ToWorkspace  VariableName=SOC_internal  SaveFormat=Timeseries  SampleTime=-1
  SOC_realtime : ToWorkspace  VariableName=SOC_realtime  SaveFormat=Timeseries  SampleTime=-1
  Saturation : Saturate  UpperLimit=inf  LowerLimit=1
  Saturation1 : Saturate  UpperLimit=Db_max  LowerLimit=Db_min
  Saturation2 : Saturate  UpperLimit=Ibat_max  LowerLimit=-Ibat_max
  Saturation3 : Saturate  UpperLimit=1  LowerLimit=0
  Saturation4 : Saturate  UpperLimit=Pref_max  LowerLimit=Pref_min
  Saturation_Dpv : Saturate  UpperLimit=Dpv_max  LowerLimit=Dpv_min
  Selector3 : Selector  InputPortWidth=6  IndexOptions=Index vector (dialog)  Indices=[1 3 5]  OutputSizes=1
  Series RLC Branch : spsSeriesRLCBranchLib/Series RLC Branch  LConnTagsString=__new0  RConnTagsString=__new0  BranchType=RL  Resistance=RLbat  Inductance=Lbat  SetiL0=on  InitialCurrent=Ibat0  Capacitance=1e-6  Setx0=off  InitialVoltage=0  Measurements=None
  Sine Wave : Sin  Amplitude=Vac_phase_peak  Frequency=2*pi*f_grid  SampleTime=Ts_mpc
  Sine Wave1 : Sin  Amplitude=Vac_phase_peak  Frequency=2*pi*f_grid  Phase=-2*pi/3  SampleTime=Ts_mpc
  Sine Wave2 : Sin  Amplitude=Vac_phase_peak  Frequency=2*pi*f_grid  Phase=2*pi/3  SampleTime=Ts_mpc
  "Sinusoidal Measurement (PLL, Three-Phase)" : eeSinusoidalMeasurementV2/Sinusoidal Measurement (PLL, Three-Phase)  InputFilter=on  InputNormalization=on  Kp_LF=1  Ki_LF=10  F0=50  Theta0=0  Ts=Ts_mpc
      settings: LibrarySourceBlock=|
      | ee_sl_lib/Measurements/Sinusoidal Measurement
      | (PLL, Three-Phase)
  "Sinusoidal Measurement (PLL, Three-Phase)1" : eeSinusoidalMeasurementV2/Sinusoidal Measurement (PLL, Three-Phase)  InputFilter=on  InputNormalization=on  Kp_LF=1  Ki_LF=10  F0=50  Theta0=0  Ts=Ts_mpc
      settings: LibrarySourceBlock=|
      | ee_sl_lib/Measurements/Sinusoidal Measurement
      | (PLL, Three-Phase)
  Step : Step  Time=0.002  SampleTime=0
  Step1 : Step  Time=0.004  SampleTime=0
  Step2 : Step  Time=0.004  SampleTime=0
  Step3 : Step  Time=0.002  SampleTime=0
  Step5 : Step  Time=0.004  SampleTime=0
  Sum{,4,7,9..10,13,15..18} (10 alike) : Sum  Inputs=|+-
  Sum{1..3,6,8,11..12,14,19,21} (10 alike) : Sum  Inputs=|++
  Sum20 : Sum  Inputs=|-+
  Sum22 : Sum  Inputs=|+--
  Sum5 : Sum  Inputs=|-+
  Switch{,1..5,7..11} (11 alike) : Switch  Criteria=u2 ~= 0  SaturateOnIntegerOverflow=off  InputSameDT=off
  Switch13 : Switch  Criteria=u2 > Threshold  SaturateOnIntegerOverflow=off  InputSameDT=off
  Switch6 : Switch  Criteria=u2 > Threshold  SaturateOnIntegerOverflow=off  InputSameDT=off
  Switch_safe_dV : Switch  Criteria=u2 ~= 0  SaturateOnIntegerOverflow=off  InputSameDT=off
  Synchronization_Reference_Select : Switch  Criteria=u2 ~= 0  SaturateOnIntegerOverflow=off  InputSameDT=off
  Three-Phase Parallel RLC Load : spsThreePhaseParallelRLCLoadLib/Three-Phase Parallel RLC Load  LConnTagsString=A|B|C  Configuration=Y (grounded)  NominalVoltage=Vac_ll  Vabc=[1e3 1e3 1e3]  Vabcp=[1e3 1e3 1e3]  NominalFrequency=f_grid  UnbalancedPower=off  ActivePower=0  InductivePower=0  CapacitivePower=Qc_filter  Pabc=[10e3 9e3 11e3]  QLabc=[100 90 110]  QCabc=[100 90 110]  Pabcp=[10e3 9e3 11e3]  QLabcp=[100 90 110]  QCabcp=[100 90 110]  Measurements=None  LoadType=constant Z
  Three-Phase Parallel RLC Load1 : spsThreePhaseParallelRLCLoadLib/Three-Phase Parallel RLC Load  LConnTagsString=A|B|C  Configuration=Y (grounded)  NominalVoltage=Vac_ll  Vabc=[1e3 1e3 1e3]  Vabcp=[1e3 1e3 1e3]  NominalFrequency=f_grid  UnbalancedPower=off  ActivePower=P_ac_base  InductivePower=0  CapacitivePower=0  Pabc=[10e3 9e3 11e3]  QLabc=[100 90 110]  QCabc=[100 90 110]  Pabcp=[10e3 9e3 11e3]  QLabcp=[100 90 110]  QCabcp=[100 90 110]  Measurements=None  LoadType=constant Z
  Three-Phase Parallel RLC Load2 : spsThreePhaseParallelRLCLoadLib/Three-Phase Parallel RLC Load  LConnTagsString=A|B|C  Configuration=Y (grounded)  NominalVoltage=Vac_ll  Vabc=[1e3 1e3 1e3]  Vabcp=[1e3 1e3 1e3]  NominalFrequency=f_grid  UnbalancedPower=off  ActivePower=P_ac_step  InductivePower=0  CapacitivePower=0  Pabc=[10e3 9e3 11e3]  QLabc=[100 90 110]  QCabc=[100 90 110]  Pabcp=[10e3 9e3 11e3]  QLabcp=[100 90 110]  QCabcp=[100 90 110]  Measurements=None  LoadType=constant Z
  Three-Phase Series RLC Branch : spsThreePhaseSeriesRLCBranchLib/Three-Phase Series RLC Branch  LConnTagsString=A|B|C  RConnTagsString=A|B|C  BranchType=RL  Resistance=Rf  Inductance=Lf  Capacitance=1e-6  Measurements=None
  Three-Phase Transformer (Two Windings) : spsThreePhaseTransformerTwoWindingsLib/Three-Phase Transformer (Two Windings)  Winding1Connection=Yg  Winding2Connection=Yg  CoreType=Three single-phase transformers  SetSaturation=off  Hysteresis=off  DataFile='hysteresis'  SetInitialFlux=off  Measurements=None  UNITS=pu  NominalPower=[ S_tr , f_grid ]  Winding1=[ V_tr_lv , 0.002 , 0.06 ]  Winding2=[ V_tr_hv , 0.002 , 0.06 ]  Rm=500  Lm=500  L0=0.5  Saturation=[ 0,0 ; 0.0024,1.2 ; 1.0,1.52 ]  InitialFluxes=[ 0.8 , -0.8 , 0.7 ]  BreakLoop=off  DiscreteSolver=Trapezoidal iterative  DataType=off  TransfoNumber=1
  Three-Phase V-I Measurement1 : spsThreePhaseVIMeasurementLib/Three-Phase V-I Measurement  VoltageMeasurement=phase-to-ground  SetLabelV=off  LabelV=Vabc  Vpu=off  VpuLL=off  CurrentMeasurement=yes  SetLabelI=off  LabelI=Iabc  Ipu=off  Pbase=100e6  Vbase=500e3  OutputType=Complex  PhasorSimulation=off  PSBequivalent=0
  Three-Phase Breaker : spsThreePhaseBreakerLib/Three-Phase Breaker  InitialState=open  SwitchA=on  SwitchB=on  SwitchC=on  SwitchTimes="[1/60  5/60]"  External=on  BreakerResistance=1e-3  SnubberResistance=1e6  SnubberCapacitance=inf  Measurements=None
  Three-Phase Breaker1 : spsThreePhaseBreakerLib/Three-Phase Breaker  InitialState=closed  SwitchA=on  SwitchB=on  SwitchC=on  SwitchTimes="[1/60  5/60]"  External=on  BreakerResistance=1e-3  SnubberResistance=1e6  SnubberCapacitance=inf  Measurements=None
  Three-Phase Breaker2 : spsThreePhaseBreakerLib/Three-Phase Breaker  InitialState=closed  SwitchA=on  SwitchB=on  SwitchC=on  SwitchTimes="[1/60  5/60]"  External=on  BreakerResistance=1e-3  SnubberResistance=1e6  SnubberCapacitance=inf  Measurements=None
  Triggered Subsystem : Subsystem  TreatAsAtomicUnit=on
  Trigonometric Function : Trigonometry  Operator=cos
  Two-Quadrant DC/DC Converter : spsTwoQuadrantDCDCConverterLib/Two-Quadrant DC//DC Converter  ModelType=Switching devices  Ron=1e-3  Rs=1e6  Cs=inf  Vforward=[0,0]  Ron_Diode=1e-3  Rs_Diode=1e6  Cs_Diode=inf  Vf_Diode=1e-3  Rs_CurrentSource=inf  Ron_ACsource=1e-3
  Unit Delay : UnitDelay  InitialCondition=Vpv0  SampleTime=Ts_mppt  HasFrameUpgradeWarning=on
  Unit Delay1 : UnitDelay  SampleTime=Ts_mppt  HasFrameUpgradeWarning=on
  Unit Delay2 : UnitDelay  InitialCondition=Dpv0  SampleTime=Ts_mppt  HasFrameUpgradeWarning=on
  Unit Delay3 : UnitDelay  SampleTime=Ts_power  HasFrameUpgradeWarning=on
  Unit Delay4 : UnitDelay  SampleTime=Ts_power  HasFrameUpgradeWarning=on
  Unit Delay7 : UnitDelay  SampleTime=Ts_mpc  HasFrameUpgradeWarning=on
  Unit Delay8 : UnitDelay  SampleTime=-1  HasFrameUpgradeWarning=on
  Unit Delay9 : UnitDelay  InitialCondition=[0;0;0]  SampleTime=Ts_mpc  HasFrameUpgradeWarning=on
  Universal Bridge : spsUniversalBridgeLib/Universal Bridge  Arms=3  SnubberResistance=1e5  SnubberCapacitance=inf  Device=IGBT / Diodes  Ron=Ron_switch  Lon=0  ForwardVoltages="[  Vf_diode  Vf_diode  ]"  ForwardVoltage=0  GTOparameters=[ 10e-6 , 20e-6 ]  IGBTparameters=[ 1e-6 , 2e-6 ]  Measurements=None  Measurements_2=None  converterType=Rectifier
  V_L_rms : ToWorkspace  VariableName=V_L_rms  SaveFormat=Timeseries  SampleTime=-1
  V_bat : ToWorkspace  VariableName=V_bat  SaveFormat=Timeseries  SampleTime=-1
  V_dc : ToWorkspace  VariableName=V_dc  SaveFormat=Timeseries  SampleTime=-1
  V_dc_REF : Constant  Value=1200
  V_grid_clarke : ToWorkspace  VariableName=V_grid_clarke  SaveFormat=Timeseries  SampleTime=-1
  V_pv : ToWorkspace  VariableName=V_pv  SaveFormat=Timeseries  SampleTime=-1
  Vabc_L : ToWorkspace  VariableName=Vabc_L  SaveFormat=Timeseries  SampleTime=-1
  Vabc_grid : ToWorkspace  VariableName=Vabc_grid  SaveFormat=Timeseries  SampleTime=-1
  Vabc_load : ToWorkspace  VariableName=Vabc_load  SaveFormat=Timeseries  SampleTime=-1
  Vf_ph_clarke : ToWorkspace  VariableName=Vf_ph_clarke  SaveFormat=Timeseries  SampleTime=-1
  Vg_pu : FromWorkspace  VariableName=GridVpu_profile  OutputAfterFinalValue=Holding final value
  Voltage Measurement : spsVoltageMeasurementLib/Voltage Measurement  PhasorSimulation=off  OutputType=Complex  PSBequivalent=0
  Voltage Measurement1 : spsVoltageMeasurementLib/Voltage Measurement  PhasorSimulation=off  OutputType=Complex  PSBequivalent=0
  Zero-Order Hold : ZeroOrderHold  SampleTime=Ts_mppt
  Zero-Order Hold1 : ZeroOrderHold  SampleTime=Ts_mppt
  Zero-Order Hold{3..16} (14 alike) : ZeroOrderHold  SampleTime=Ts_mpc
  Zero-Order Hold2 : ZeroOrderHold  SampleTime=Ts_bat_ctrl
  battCmd : ToWorkspace  VariableName=battCmd  SaveFormat=Timeseries  SampleTime=-1
  control_enable : ManualSwitch
  grid_Iabc.log : ToWorkspace  VariableName=grid_Iabc  SaveFormat=Timeseries  SampleTime=-1
  grid_VI : spsThreePhaseVIMeasurementLib/Three-Phase V-I Measurement  VoltageMeasurement=phase-to-ground  SetLabelV=off  LabelV=Vabc  Vpu=off  VpuLL=off  CurrentMeasurement=yes  SetLabelI=off  LabelI=Iabc  Ipu=off  Pbase=100e6  Vbase=500e3  OutputType=Complex  PhasorSimulation=off  PSBequivalent=0
  log_P_grid_threephase : ToWorkspace  VariableName=P_grid_threephase  SaveFormat=Timeseries  SampleTime=-1
  log_Q_grid_threephase : ToWorkspace  VariableName=Q_grid_threephase  SaveFormat=Timeseries  SampleTime=-1
  powergui : sps_lib/powergui  Priority=1  SimulationMode=Discrete  SampleTime=Ts_power  frequency=60  Iterations=50  frequencyindice=0  Pbase=100e6  ErrMax=1e-4  UnitsV=kV  UnitsW=MW  buscounter=0  FunctionMessages=off  echomessages=off  EnableUseOfTLC=off  CurrentSourceSwitches=off  DisableSnubberDevices=off  DisableRonSwitches=off  DisableVfSwitches=off  DisplayEquations=off  AutomaticDiscreteSolvers=off  SolverType=Tustin/Backward Euler (TBE)  Interpol=off  ExternalGateDelay=off  methode=off  Ts=100  x0status=blocks  SPID=on  SwTol=0  HookPort=off  NonlinearTolerance=1e-4  nMaxIteration=100  ContinueOnMaxIteration=off  RestoreLinks=warning  ResistiveCurrentMeasurement=off  Frange=[0:2:500]  Ylog=off  Xlog=on  ShowGrid=off  save=off  variable=ZData  structure=0  ZoomFFT=off  StartTime=0.0  cycles=1  DisplayStyle=1  fundamental=60  FreqAxis=off  MaxFrequency=1000  frequencyindicesteady=1  RmsSteady=1  display=off
  stateIndex_MPPC : ToWorkspace  VariableName=stateIndex_MPPC  SaveFormat=Timeseries  SampleTime=-1
  stateindex_mpvc : ToWorkspace  VariableName=stateindex_mpvc  SaveFormat=Timeseries  SampleTime=-1
  sync : Step  Time=T_sync  SampleTime=Ts_mpc
  sync1 : Step  Time=T_sync  SampleTime=Ts_mpc
  wires:
  From Workspace2/1 -> PV Array/1
  Constant1/1 -> PV Array/2
  Current Measurement/1 -> [I_pv]
  Voltage Measurement1/1 -> [V_pv]
  [V_pv] -> Product/1
  [I_pv] -> Product/2
  Product/1 -> Moving Average1/1
  [V_pv] -> V_pv/1
  [I_pv] -> I_pv/1
  Voltage Measurement/1 -> [V_dc]
  [V_dc] -> V_dc/1
  PWM Generator (DC-DC)/1 -> Pv_boost/1
  Step/1 -> Pv_input_isolator/1
  Step1/1 -> DC_output_isolator/1
  Constant3/1 -> Pv_boost/2
  [V_pv] -> Zero-Order Hold/1
  [I_pv] -> Zero-Order Hold1/1
  Zero-Order Hold/1 -> [Vk]  "Vk"
  Zero-Order Hold1/1 -> [Ik]  "Ik"
  [Vk] -> Unit Delay/1
  [Ik] -> Unit Delay1/1
  Unit Delay/1 -> [V_k_1]  "Vk-1"
  Unit Delay1/1 -> [I_k_1]  "Ik-1"
  [Vk] -> Sum/1
  [V_k_1] -> Sum/2
  Sum/1 -> [dV]  "dV"
  [Ik] -> Sum4/1
  [I_k_1] -> Sum4/2
  Sum4/1 -> [dI]  "dI"
  [dV] -> Abs/1
  Abs/1 -> Compare To Constant1/1
  Constant4/1 -> Switch_safe_dV/1
  [dV] -> Switch_safe_dV/3
  Switch_safe_dV/1 -> [safe_dV]  "safe_dV"
  [Vk] -> Saturation/1
  Saturation/1 -> [safe_Vk]  "safe_Vk"
  [dI] -> Divide1/1
  [safe_dV] -> Divide1/2
  [safe_Vk] -> Divide2/2
  [Ik] -> Divide2/1
  Divide1/1 -> Sum3/1
  Divide2/1 -> Sum3/2
  Sum3/1 -> [Inc]
  [Inc] -> Compare To Constant/1
  [Inc] -> Compare To Constant2/1
  Compare To Constant/1 -> Switch/2
  Constant5/1 -> Product1/1
  Constant6/1 -> Product1/2
  Product1/1 -> Switch/1
  Switch1/1 -> Switch/3
  Compare To Constant2/1 -> Switch1/2
  Constant8/1 -> Switch1/1
  Constant9/1 -> Switch1/3
  Switch/1 -> [D_PV_STEP_NORMAL]
  Product2/1 -> Switch2/1
  Switch3/1 -> Switch2/3
  Constant11/1 -> Switch3/1
  Constant7/1 -> Product2/1
  Switch2/1 -> [D_PV_STEP_dV0]
  Constant10/1 -> Product2/2
  [dI] -> Compare To Constant4/1
  [dI] -> Compare To Constant3/1
  Constant12/1 -> Switch3/3
  Compare To Constant4/1 -> Switch3/2
  Compare To Constant3/1 -> Switch2/2
  [dV_small] -> Switch4/2
  [D_PV_STEP_dV0] -> Switch4/1
  [D_PV_STEP_NORMAL] -> Switch4/3
  Switch4/1 -> Sum1/1  "dD"
  Unit Delay2/1 -> Sum1/2
  Sum1/1 -> Saturation_Dpv/1
  Saturation_Dpv/1 -> Unit Delay2/1, Switch7/3
  Constant2/1 -> Manual Switch/2
  Manual Switch/1 -> PWM Generator (DC-DC)/1
  Compare To Constant1/1 -> [dV_small]  "dV_small"
  [dV_small] -> Switch_safe_dV/2
  [Dpv] -> Dpv/1  "Dpv"
  [I_Rdc1] -> Sum2/1
  [I_Rdc2] -> Sum2/2
  Sum2/1 -> Idc_load/1, [Idc_load]  "Idc_load"
  [Idc_load] -> Product3/2
  [V_dc] -> Product3/1
  Product3/1 -> Moving Average2/1  "P_DC"
  Current Measurement1/1 -> [I_Rdc1]  "I_Rdc1"
  Current Measurement2/1 -> [I_Rdc2]  "I_Rdc2"
  Product4/1 -> P_DC_load1/1  "P_DC_load1"
  [I_Rdc1] -> Product4/2
  [V_dc] -> Product5/1
  [I_Rdc2] -> Product5/2
  Product5/1 -> P_DC_load2/1  "P_DC_load2"
  PWM Generator (DC-DC)1/1 -> [PWM_bat]  "PWM_bat"
  [PWM_bat] -> AND/1
  [PWM_bat] -> Unit Delay3/1
  Unit Delay3/1 -> AND/2
  AND/1 -> [gate_lower]
  [PWM_bat] -> NOT/1
  NOT/1 -> AND1/1
  [PWM_bat] -> NOT1/1
  NOT1/1 -> Unit Delay4/1
  Unit Delay4/1 -> AND1/2
  AND1/1 -> [gate_upper]
  [gate_upper] -> Mux/1
  [gate_lower] -> Mux/2
  Mux/1 -> Data Type Conversion/1
  Constant14/1 -> Two-Quadrant DC/DC Converter/2
  Data Type Conversion/1 -> [gate_bat]
  [gate_bat] -> Two-Quadrant DC/DC Converter/1
  Current Measurement3/1 -> [I_bat], I_bat/1
  Battery/1 -> [Battery]
  [Battery] -> Bus Selector/1
  Bus Selector/2 -> I_sourcebat/1  "<Current (A)>"
  Bus Selector/3 -> SOC_internal/1  "<SOC (%)>"
  Step2/1 -> Battery DC Isolator/1
  Step3/1 -> Battery Isolato/1
  Discrete PID Controller/1 -> Sum6/1
  Constant16/1 -> Sum6/2
  Sum6/1 -> D_bat/1, Saturation1/1
  Sum5/1 -> Discrete PID Controller/1
  Zero-Order Hold2/1 -> Sum5/1
  Saturation1/1 -> [D_bat]  "D_bat"
  Manual Switch1/1 -> PWM Generator (DC-DC)1/1
  [D_bat] -> Manual Switch1/1
  Constant13/1 -> Manual Switch1/2
  [I_bat] -> Moving Average/1
  Moving Average/1 -> [I_bat_mean], I_bat_mean/1, Zero-Order Hold2/1
  [I_bat_mean] -> I_bat to SOC/1
  I_bat to SOC/1 -> Discrete-Time Integrator/1
  V_dc_REF/1 -> Sum7/1
  [V_dc] -> Sum7/2
  [grid_state] -> Switch5/2
  Switch5/1 -> [I_ref]
  [I_ref_EMS] -> Switch5/1
  From Workspace/1 -> DC_load1/1
  From Workspace1/1 -> DC_load2/1
  Constant26/1 -> Max/2
  Relational Operator1/1 -> Switch10/2
  [SOC_realtime] -> Relational Operator1/1
  Constant20/1 -> Relational Operator1/2
  [SOC_realtime] -> Relational Operator3/1
  Constant23/1 -> Relational Operator3/2
  Relational Operator3/1 -> Switch11/2
  [I_ref] -> Max1/1
  Constant27/1 -> Max1/2
  Max1/1 -> Switch11/1
  [I_ref] -> Switch11/3
  Max/1 -> Switch10/1
  [I_ref_protected] -> Sum5/2
  Switch11/1 -> Switch10/3, Max/1
  [I_ref] -> MATLAB Function/1(Iref)
  Constant24/1 -> MATLAB Function/4(SOC_max)
  Constant21/1 -> MATLAB Function/3(SOC_min)
  Step5/1 -> Breaker/1
  LC_VI/1 -> [Vabc_L]
  LC_VI/2 -> [Iabc_L]
  Three-Phase V-I Measurement1/1 -> [Vabc_load]
  Three-Phase V-I Measurement1/2 -> [Iabc_load]
  [Vabc_L] -> Vabc_L/1
  [Iabc_L] -> Iabc_L/1
  [Vabc_load] -> Vabc_load/1
  [Iabc_load] -> Iabc_load/1
  [Vabc_L] -> RMS/1
  RMS/1 -> V_L_rms/1
  [Vabc_L] -> Gain1/1
  [Vf_ph_clarke] -> Demux/1
  [Iabc_L] -> Gain3/1
  [If_clarke] -> Demux1/1
  [V_a_clarke] -> Product6/1
  [V_b_clarke] -> Product7/1
  Product6/1 -> Sum8/1
  Product7/1 -> Sum8/2
  Product9/1 -> Sum9/2
  Product8/1 -> Sum9/1
  [V_b_clarke] -> Product8/1
  [I_a_clarke] -> Product6/2
  [I_b_clarke] -> Product7/2
  [I_a_clarke] -> Product8/2
  [V_a_clarke] -> Product9/1
  [I_b_clarke] -> Product9/2
  Sum8/1 -> Gain4/1
  Sum9/1 -> Gain5/1
  [Iabc_load] -> Gain6/1
  Demux1/1 -> [I_a_clarke]
  Demux1/2 -> [I_b_clarke]
  [I_load_clarke] -> I_load_clarke/1
  [If_clarke] -> If_clarke/1
  [Vf_ph_clarke] -> Vf_ph_clarke/1
  Constant28/1 -> MATLAB Function1/6(Ad)
  Constant29/1 -> MATLAB Function1/7(Bd)
  Constant25/1 -> MATLAB Function1/8(lambda_sw)
  Sine Wave1/1 -> Mux2/2
  Sine Wave2/1 -> Mux2/3
  Sine Wave/1 -> Mux2/1
  Mux2/1 -> [Vc_abc_ref]
  Gain7/1 -> Zero-Order Hold7/1
  MATLAB Function1/1(gates) -> [gates_mpvc]
  [previousState_actual] -> MATLAB Function1/9(previousState)
  [gates_ac_enable] -> Universal Bridge/1
  Gain6/1 -> Zero-Order Hold8/1
  Zero-Order Hold8/1 -> [I_load_clarke]
  [I_load_clarke] -> MATLAB Function1/4(IL_ab)
  Gain3/1 -> Zero-Order Hold9/1
  Zero-Order Hold9/1 -> [If_clarke]
  Zero-Order Hold10/1 -> [Vf_ph_clarke]
  Gain1/1 -> Zero-Order Hold10/1
  Demux/1 -> [V_a_clarke]
  Demux/2 -> [V_b_clarke]
  [Vf_ph_clarke] -> MATLAB Function1/2(Vc_ab)
  [If_clarke] -> MATLAB Function1/3(If_ab)
  Product11/1 -> Data Type Conversion1/1
  Data Type Conversion1/1 -> [gates_ac_enable]
  MATLAB Function1/2(stateIndex) -> stateindex_mpvc/1
  MATLAB Function1/3(Jmin) -> Jmin_mpvc/1
  [V_dc] -> Zero-Order Hold3/1
  Zero-Order Hold3/1 -> MATLAB Function1/1(Vdc)
  grid_VI/1 -> [grid_Vabc]
  [grid_Vabc] -> Synchronization_Reference_Select/1
  Zero-Order Hold7/1 -> [Vc_ab_ref]
  [Vc_ab_ref] -> MATLAB Function1/5(Vref_ab)
  [Vc_abc_ref] -> Synchronization_Reference_Select/3
  sync/1 -> Synchronization_Reference_Select/2
  Synchronization_Reference_Select/1 -> [Vref_abc]
  [Vref_abc] -> Gain7/1
  [grid_Vabc] -> Vabc_grid/1
  GridConnectEnable/1 -> AND2/1
  [closePermit] -> AND2/2
  grid_VI/2 -> [grid_Iabc]
  [grid_Iabc] -> grid_Iabc.log/1
  Vg_pu/1 -> Bias/1
  Bias/1 -> Gain/1
  Gain/1 -> Log_Qref_Command/1, [Q_ref]
  [gates_mpvc] -> Switch6/3
  MATLAB Function2/1(gates) -> [gates_mppv]
  [gates_mppv] -> Switch6/1
  [grid_state] -> Switch6/2
  Switch6/1 -> Product11/1
  Constant32/1 -> control_enable/2
  Constant30/1 -> control_enable/1
  control_enable/1 -> Product11/2
  [V_dc] -> Zero-Order Hold4/1
  Zero-Order Hold4/1 -> MATLAB Function2/1(Vdc)
  Gain2/1 -> Zero-Order Hold5/1
  [grid_Vabc] -> Gain2/1
  Zero-Order Hold5/1 -> V_grid_clarke/1, [V_grid_clarke]
  [V_grid_clarke] -> MATLAB Function2/2(Vg_ab)
  [P_MPPC] -> Zero-Order Hold6/1
  Zero-Order Hold6/1 -> MATLAB Function2/3(P)
  [Q_MPPC] -> Zero-Order Hold11/1
  Zero-Order Hold11/1 -> MATLAB Function2/4(Q)
  [Q_ref] -> Zero-Order Hold12/1
  Zero-Order Hold12/1 -> MATLAB Function2/6(Qref)
  [P_ref] -> Zero-Order Hold13/1
  Zero-Order Hold13/1 -> MATLAB Function2/5(Pref)
  Constant33/1 -> MATLAB Function2/7(Ts)
  Constant34/1 -> MATLAB Function2/8(Lf)
  Constant36/1 -> MATLAB Function2/9(Rf)
  Constant35/1 -> MATLAB Function2/10(omega)
  [previousState_actual] -> MATLAB Function2/14(previousState)
  Constant37/1 -> MATLAB Function2/13(lambda_sw)
  Constant38/1 -> MATLAB Function2/11(Pbase)
  Constant39/1 -> MATLAB Function2/12(Qbase)
  [P_pv] -> EMS_flowchart/1(Ppv)
  [P_dc] -> EMS_flowchart/3(Pdc)
  [Pf_threephase] -> EMS_flowchart/2(Pac)
  [grid_state] -> Data Type Conversion2/1
  Data Type Conversion2/1 -> EMS_flowchart/5(GridConnected)
  EMS_flowchart/1(Ibat_ref) -> [I_ref_EMS]
  EMS_flowchart/2(battCmd) -> battCmd/1
  [offMPPT] -> Switch7/2
  [load_Shed] -> NOT2/1
  NOT2/1 -> Three-Phase Breaker1/1
  Moving Average1/1 -> P_pv/1, [P_pv]
  Moving Average2/1 -> [P_dc], P_DC/1
  Gain4/1 -> Moving Average3/1
  Moving Average3/1 -> Pf_threephase/1, [Pf_threephase]
  Gain5/1 -> Moving Average4/1
  Moving Average4/1 -> [Qf_threephase], Qf_threephase/1
  ProtectionLogic/1(loadShed) -> [load_Shed]
  EMS_flowchart/3(ShedReq) -> [ShedReq]
  EMS_flowchart/4(offMPPTReq) -> [offMPPTReq]
  [ShedReq] -> ProtectionLogic/1(ShedReq)
  [offMPPTReq] -> ProtectionLogic/2(offMPPTReq)
  [SOC_realtime] -> ProtectionLogic/3(SOC)
  [Ig_b_clarke] -> Product13/2
  Gain8/1 -> Moving Average5/1
  [Ig_a_clarke] -> Product12/2
  Product12/1 -> Sum11/1
  Product13/1 -> Sum11/2
  Moving Average5/1 -> log_P_grid_threephase/1, [P_grid_threephase]
  Sum11/1 -> Gain8/1
  [Vg_b_clarke] -> Product13/1
  [Vg_a_clarke] -> Product12/1
  Zero-Order Hold14/1 -> [V_grid_ph_clarke]
  Gain9/1 -> Zero-Order Hold14/1
  [grid_Vabc] -> Gain9/1
  [V_grid_ph_clarke] -> Demux2/1
  Demux2/1 -> [Vg_a_clarke]
  Demux2/2 -> [Vg_b_clarke]
  Gain10/1 -> Zero-Order Hold15/1
  Zero-Order Hold15/1 -> [I_grid_ph_clarke]
  [grid_Iabc] -> Gain10/1
  Demux3/2 -> [Ig_b_clarke]
  Demux3/1 -> [Ig_a_clarke]
  Product14/1 -> Sum13/1
  Moving Average6/1 -> log_Q_grid_threephase/1, [Q_grid_threephase]
  Sum13/1 -> Gain11/1
  Gain11/1 -> Moving Average6/1
  Product15/1 -> Sum13/2
  [I_grid_ph_clarke] -> Demux3/1
  [Vg_b_clarke] -> Product14/1
  [Ig_a_clarke] -> Product14/2
  [Vg_a_clarke] -> Product15/1
  [Ig_b_clarke] -> Product15/2
  [grid_Iabc] -> Iabc_grid/1
  Product19/1 -> Sum15/2
  Sum15/1 -> Gain12/1
  [Vg_b_clarke] -> Product17/1
  [Vg_b_clarke] -> Product18/1
  [Vg_a_clarke] -> Product19/1
  [I_b_clarke] -> Product17/2
  [I_a_clarke] -> Product16/2
  Product18/1 -> Sum15/1
  Product16/1 -> Sum14/1
  Product17/1 -> Sum14/2
  [Vg_a_clarke] -> Product16/1
  Sum14/1 -> Gain13/1
  [I_a_clarke] -> Product18/2
  Gain13/1 -> [P_MPPC], Moving Average9/1
  [I_b_clarke] -> Product19/2
  Gain12/1 -> [Q_MPPC], Moving Average10/1
  [grid_Vabc] -> Sum16/1
  [Vabc_L] -> Sum16/2
  Sum16/1 -> Demux4/1
  Demux4/1 -> RMS Measurement/1
  Demux4/2 -> RMS Measurement1/1
  Demux4/3 -> RMS Measurement2/1
  RMS Measurement/1 -> Mux3/1
  RMS Measurement1/1 -> Mux3/2
  RMS Measurement2/1 -> Mux3/3
  Mux3/1 -> MinMax1/1
  MinMax1/1 -> Compare To Constant5/1
  Compare To Constant5/1 -> AND3/1
  [grid_Vabc] -> "Sinusoidal Measurement (PLL, Three-Phase)"/1
  [Vabc_L] -> "Sinusoidal Measurement (PLL, Three-Phase)1"/1
  "Sinusoidal Measurement (PLL, Three-Phase)1"/1 -> Sum17/2
  "Sinusoidal Measurement (PLL, Three-Phase)"/1 -> Sum17/1
  "Sinusoidal Measurement (PLL, Three-Phase)"/2 -> Sum18/1
  "Sinusoidal Measurement (PLL, Three-Phase)1"/2 -> Sum18/2
  Sum17/1 -> Abs2/1
  Abs2/1 -> Compare To Constant6/1
  Compare To Constant6/1 -> AND3/2
  Sum18/1 -> Trigonometric Function/1
  Trigonometric Function/1 -> Compare To Constant7/1
  Compare To Constant7/1 -> AND3/3
  Unit Delay7/1 -> Sum19/2  "Tgood_prev"
  Constant17/1 -> Sum19/1
  Sum19/1 -> Switch8/1
  [BasicSync_OK] -> Switch8/2
  Constant22/1 -> Switch8/3
  Switch8/1 -> Compare To Constant8/1, [Tgood]
  [Tgood] -> Unit Delay7/1
  Compare To Constant8/1 -> [closePermit]
  AND2/1 -> S-R Flip-Flop/1
  Constant40/1 -> S-R Flip-Flop/2
  S-R Flip-Flop/1 -> [GridConnected]
  [GridConnected] -> [grid_state], Three-Phase Breaker/1
  [grid_state] -> P_ref  occured/Enable
  P_ref  occured/1(P_ref) -> Product21/2
  [grid_state] -> Triggered Subsystem/Trigger
  [P_MPPC] -> Zero-Order Hold16/1
  Zero-Order Hold16/1 -> Triggered Subsystem/1(P_meas)
  [grid_state] -> Switch9/2
  Constant41/1 -> Sum12/2
  Sum12/1 -> Saturation3/1
  Saturation3/1 -> Switch9/1
  Constant42/1 -> Switch9/3
  Unit Delay8/1 -> Sum12/1
  Switch9/1 -> Sum20/1, Unit Delay8/1, Product21/1  "alpha"
  Sum20/1 -> Product20/2
  Triggered Subsystem/1(P0) -> Product20/1
  Constant43/1 -> Sum20/2
  Product20/1 -> Sum21/1
  Product21/1 -> Sum21/2
  Sum21/1 -> Saturation4/1
  [V_dc] -> P_ref  occured/1(V_DC)
  Saturation4/1 -> Log_Pref_Command/1, [P_ref]
  [grid_state] -> Switch13/2
  [gates_mppv] -> Switch13/1
  [gates_mpvc] -> Switch13/3
  Unit Delay9/1 -> [previousState_actual]
  Selector3/1 -> Unit Delay9/1
  Switch13/1 -> Selector3/1
  AND3/1 -> AND4/1
  AND4/1 -> [BasicSync_OK]
  sync1/1 -> AND4/2
  MATLAB Function2/2(stateIndex) -> stateIndex_MPPC/1
  MATLAB Function2/3(Jmin) -> Jmin_MPPC/1
  Moving Average9/1 -> "P_MPPC "/1
  Moving Average10/1 -> Q_MPPC/1
  AC_load_Step/1 -> Three-Phase Breaker2/1
  Bus Selector/1 -> V_bat/1, [V_bat]  "<Voltage (V)>"
  [I_bat_mean] -> Product10/1
  [V_bat] -> Product10/2
  Product10/1 -> P_bat/1
  Discrete-Time Integrator/1 -> SOC_realtime/1, [SOC_realtime]
  [SOC_realtime] -> MATLAB Function/2(SOC)
  RMS1/1 -> Iabc_L_rms/1
  [Iabc_L] -> RMS1/1
  [SOC_realtime] -> EMS_flowchart/4(SOC)
  PI_voltage/1 -> Sum10/1, I_ref_raw/1
  Sum10/1 -> Saturation2/1
  [I_ref_EMS] -> I_ref_ems/1
  Saturation2/1 -> Switch5/3
  Sum7/1 -> PI_voltage/1
  [Iabc_load] -> Dot Product/1
  [Vabc_load] -> Dot Product/2
  [P_pv] -> Sum22/1
  [P_dc] -> Sum22/2
  Dot Product/1 -> Sum22/3
  Sum22/1 -> Divide/1
  Constant/1 -> Divide/2
  Divide/1 -> [I_forward]
  [I_forward] -> Sum10/2
  [Dpv] -> Manual Switch/1  "Dpv"
  A_phase/1 -> Mux1/1
  B_phase/1 -> Mux1/2
  C_phase/1 -> Mux1/3
  Mux1/1 -> PWM Generator (2-Level)/1
  Switch7/1 -> PV_Duty_Bumpless_Transfer/1
  PV_Duty_Bumpless_Transfer/1 -> [Dpv]
  [V_dc] -> PV_Curtail_Protection/2(Vdc), PV_Curtail_Duty_Controller/1(Vdc), Product4/1
  PV_Curtail_Duty_Controller/1(Dpv_Curtail) -> Switch7/1
  ProtectionLogic/2(offMPPT) -> PV_Curtail_Protection/1(Protection_OffMPPT)
  MATLAB Function/1(Iout) -> I_ref_protected/1, [I_ref_protected], PV_Curtail_Protection/3(Ibat_Reference)
  PV_Curtail_Protection/1(OffMPPT_Final) -> [offMPPT]
  connections:
  Voltage Measurement/LConn1 -- Current Measurement2/LConn1 -- Battery DC Isolator/LConn1 -- Current Measurement1/LConn1 -- Breaker/RConn1 -- DC_output_isolator/RConn1 -- Cdc/LConn1
  PV Array/RConn1 -- C_pv/LConn1 -- Voltage Measurement1/LConn1 -- Current Measurement/LConn1
  Voltage Measurement1/LConn2 -- Universal Bridge/RConn2 -- Battery/LConn2 -- Two-Quadrant DC/DC Converter/RConn2 -- DC_load2/RConn1 -- DC_load1/RConn1 -- Voltage Measurement/LConn2 -- Cdc/RConn1 -- Pv_boost/RConn2 -- C_pv/RConn1 -- PV Array/RConn2
  L_pv/LConn1 -- Current Measurement/RConn1
  Pv_input_isolator/LConn1 -- L_pv/RConn1
  Pv_input_isolator/RConn1 -- Pv_boost/LConn1
  DC_output_isolator/LConn1 -- Pv_boost/RConn1
  Current Measurement1/RConn1 -- DC_load1/LConn1
  Current Measurement2/RConn1 -- DC_load2/LConn1
  Battery Isolato/RConn1 -- Series RLC Branch/RConn1
  Battery DC Isolator/RConn1 -- Two-Quadrant DC/DC Converter/RConn1
  Two-Quadrant DC/DC Converter/LConn1 -- Battery Isolato/LConn1
  Current Measurement3/RConn1 -- Series RLC Branch/LConn1
  Current Measurement3/LConn1 -- Battery/LConn1
  Universal Bridge/RConn1 -- Breaker/LConn1
  Three-Phase Series RLC Branch/LConn1 -- Universal Bridge/LConn1
  Universal Bridge/LConn2 -- Three-Phase Series RLC Branch/LConn2
  Universal Bridge/LConn3 -- Three-Phase Series RLC Branch/LConn3
  LC_VI/RConn1 -- Three-Phase V-I Measurement1/LConn1 -- Three-Phase Breaker/LConn1 -- Three-Phase Parallel RLC Load/LConn1
  LC_VI/RConn2 -- Three-Phase V-I Measurement1/LConn2 -- Three-Phase Breaker/LConn2 -- Three-Phase Parallel RLC Load/LConn2
  LC_VI/RConn3 -- Three-Phase V-I Measurement1/LConn3 -- Three-Phase Breaker/LConn3 -- Three-Phase Parallel RLC Load/LConn3
  LC_VI/LConn1 -- Three-Phase Series RLC Branch/RConn1
  LC_VI/LConn2 -- Three-Phase Series RLC Branch/RConn2
  LC_VI/LConn3 -- Three-Phase Series RLC Branch/RConn3
  grid_VI/LConn1 -- Three-Phase Breaker/RConn1
  grid_VI/LConn2 -- Three-Phase Breaker/RConn2
  grid_VI/LConn3 -- Three-Phase Breaker/RConn3
  Three-Phase Transformer (Two Windings)/LConn1 -- grid_VI/RConn1
  Three-Phase Transformer (Two Windings)/LConn2 -- grid_VI/RConn2
  Three-Phase Transformer (Two Windings)/LConn3 -- grid_VI/RConn3
  Three-Phase V-I Measurement1/RConn2 -- Three-Phase Breaker2/LConn2 -- Three-Phase Breaker1/LConn2
  Three-Phase V-I Measurement1/RConn3 -- Three-Phase Breaker1/LConn3 -- Three-Phase Breaker2/LConn3
  Three-Phase Breaker1/LConn1 -- Three-Phase Breaker2/LConn1 -- Three-Phase V-I Measurement1/RConn1
  Three-Phase Parallel RLC Load1/LConn3 -- Three-Phase Breaker1/RConn3
  Three-Phase Parallel RLC Load1/LConn1 -- Three-Phase Breaker1/RConn1
  Three-Phase Parallel RLC Load1/LConn2 -- Three-Phase Breaker1/RConn2
  Three-Phase Parallel RLC Load2/LConn3 -- Three-Phase Breaker2/RConn3
  Three-Phase Parallel RLC Load2/LConn2 -- Three-Phase Breaker2/RConn2
  Three-Phase Parallel RLC Load2/LConn1 -- Three-Phase Breaker2/RConn1
  Grid_Programmable_Voltage_Source/LConn1 -- Grid_Source_Ground/LConn1
  Grid_Programmable_Voltage_Source/RConn1 -- Grid_Equivalent_RL/LConn1
  Grid_Equivalent_RL/RConn1 -- Three-Phase Transformer (Two Windings)/RConn1
  Grid_Programmable_Voltage_Source/RConn2 -- Grid_Equivalent_RL/LConn2
  Grid_Equivalent_RL/RConn2 -- Three-Phase Transformer (Two Windings)/RConn2
  Grid_Programmable_Voltage_Source/RConn3 -- Grid_Equivalent_RL/LConn3
  Grid_Equivalent_RL/RConn3 -- Three-Phase Transformer (Two Windings)/RConn3
